simulink model "sim_tnse_2024_pos_ctrl"  (R2020a)
settings: Solver=ode4  StartTime=0.0  StopTime=30.0  FixedStep=0.01  RelTol=1e-3
values from neighbouring files (symbols this model uses):
  alfa_theta = 20    [init_tnse_2024_pos_ctrl.m]
  c1 = diag( [ 150.0, 120.0, 120.0 ] )    [init_tnse_2024_pos_ctrl.m]
  c1_diff_sigma_bar_v = diag([25; 30; 20])    [init_tnse_2024_pos_ctrl.m]
  c1v = diag([5.8; 6.5; 6.5])    [init_tnse_2024_pos_ctrl.m]
  c2 = diag( [ 80.0, 50.0, 50.0 ] )    [init_tnse_2024_pos_ctrl.m]
  c2_diff_sigma_bar_v = diag([50; 50; 10])    [init_tnse_2024_pos_ctrl.m]
  c2v = diag([5.8; 6.5; 6.5])    [init_tnse_2024_pos_ctrl.m]
  c3_diff_sigma_bar_v = diag([15; 15; 10])    [init_tnse_2024_pos_ctrl.m]
  c3v = diag([4.8; 6.4; 6.0])    [init_tnse_2024_pos_ctrl.m]
  dp_aa_t = 0.2 * ones(3, 5) + ( 1.0 - 0.2 ) * rand(3, 5)    [init_tnse_2024_pos_ctrl.m]
  dp_ff_t = [ 0.4 * ones(1, 5) + ( 1.0 - 0.4 ) * rand(1, 5);                      0.4 * ones(1, 5) + ( 1.0 - 0.4 ) * rand(1, 5);                      0.2 * ones(1, 5) + ( 0.6 - 0.2 ) * rand(1, 5) ]    [init_tnse_2024_pos_ctrl.m]
  dp_phi_t = ( - pi / 2 ) * ones(3, 5) + ( pi / 2 - ( - pi / 2 ) ) * rand(3, 5)    [init_tnse_2024_pos_ctrl.m]
  eps0 = [0.05; 0.01; 0.01]    [init_tnse_2024_pos_ctrl.m]
  etai_0 = zeros(3,5)    [init_tnse_2024_pos_ctrl.m]
  kai0 = [15; 10; 10]    [init_tnse_2024_pos_ctrl.m]
  kai_1_t = 0.02    [init_tnse_2024_pos_ctrl.m]
  kai_3_t = 0.1    [init_tnse_2024_pos_ctrl.m]
  ksii_0 = zeros(3,5)    [init_tnse_2024_pos_ctrl.m]
  lam0 = [15; 10; 10]    [init_tnse_2024_pos_ctrl.m]
  Lamd_diff_sigma_bar_v = 0.5    [init_tnse_2024_pos_ctrl.m]
  mass_i = zeros(1,NF)    [init_tnse_2024_pos_ctrl.m]
  Mii = diag([1;0;0;0;1])    [init_tnse_2024_pos_ctrl.m]
  pos0 = zeros(3, 1)    [init_tnse_2024_pos_ctrl.m]
  PZ0 = P0(3)    [init_tnse_2024_pos_ctrl.m]
  PZ1 = 10    [init_tnse_2024_pos_ctrl.m]
  Qci_init = repmat([1;0;0;0],1,NF)    [init_tnse_2024_pos_ctrl.m]
  R0 = 4    [init_tnse_2024_pos_ctrl.m]
  R1 = 8    [init_tnse_2024_pos_ctrl.m]
  Rx2 = 10    [init_tnse_2024_pos_ctrl.m]
  Ry2 = 6    [init_tnse_2024_pos_ctrl.m]
  Rz2 = 4    [init_tnse_2024_pos_ctrl.m]
  sat_sr_low = [-30, -30, -30]    [init_tnse_2024_pos_ctrl.m]
  sat_sr_up = [30, 30, 30]    [init_tnse_2024_pos_ctrl.m]
  T0 = 0    [init_tnse_2024_pos_ctrl.m]
  T1 = tseq1    (= 10)    [init_tnse_2024_pos_ctrl.m]
  T12 = tseq1 + tseq12    (= 20)    [init_tnse_2024_pos_ctrl.m]
  T2 = tseq1 + tseq12 + tseq2    (= 30)    [init_tnse_2024_pos_ctrl.m]
  theta0 = ( 2 / 5 ) * pi    (= 1.25663706144)    [init_tnse_2024_pos_ctrl.m]
  vel0 = zeros(3, 1)    [init_tnse_2024_pos_ctrl.m]
  Wij = [0,0,1,0,0;              0,0,1,1,0;              1,0,0,0,1;              0,1,1,0,0;              0,0,1,0,0]    [init_tnse_2024_pos_ctrl.m]
  X1 = 8    [init_tnse_2024_pos_ctrl.m]
  X2 = 2    [init_tnse_2024_pos_ctrl.m]
  X3 = 3    [init_tnse_2024_pos_ctrl.m]
  Y1 = 10    [init_tnse_2024_pos_ctrl.m]
  Y2 = 2    [init_tnse_2024_pos_ctrl.m]
  Y3 = 4    [init_tnse_2024_pos_ctrl.m]
  Z1 = 4    [init_tnse_2024_pos_ctrl.m]
  Z2 = -6    [init_tnse_2024_pos_ctrl.m]
  Z3 = 2    [init_tnse_2024_pos_ctrl.m]
  zeta_diff_sigma_bar_v = 0.08    [init_tnse_2024_pos_ctrl.m]
undefined symbols (not defined in the file or in its folder): cal_frac_squ, p_alfav1, p_alfav2, q_alfav1, q_alfav2
(part 1 of 4)
settings Model: Creator=zzy  LastModifiedBy=Hershey.A
settings DataIOCC: ReturnWorkspaceOutputs=off
settings DebuggingCC: ArithmeticOperatorsInVariantConditions=warning
settings SFSimCC: SimUseLocalCustomCode=off  CustomCodeUndefinedFunction=UseInterfaceOnly
settings RTWCC: RTWUseLocalCustomCode=off

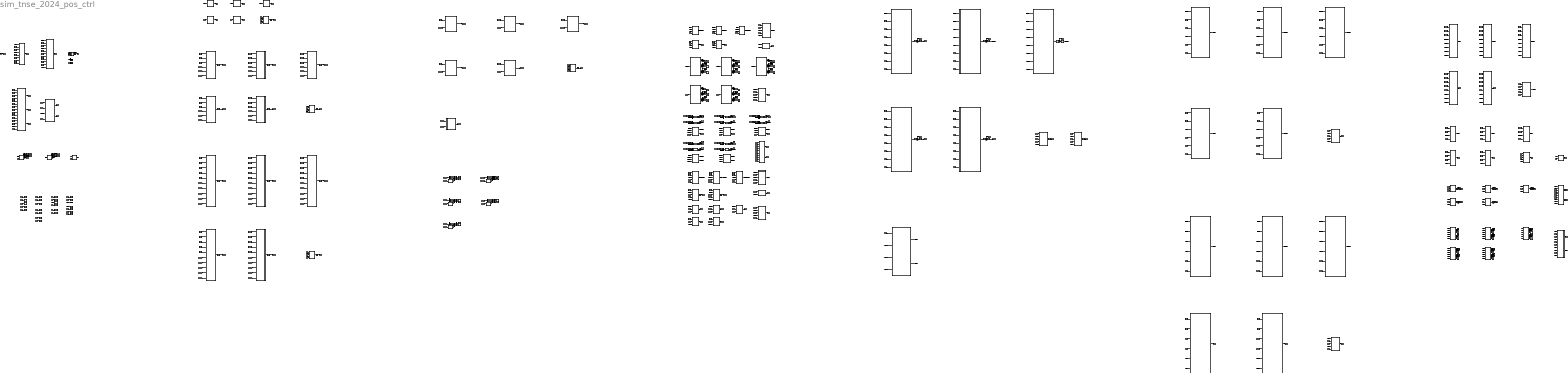
== system sim_tnse_2024_pos_ctrl ==
  Clock : Clock
  Constant{,3,6,9,14,17,22,27,32,37} (10 alike) : Constant  Value=eps0
  Constant{1,4,7,10,12,18,23,28,33,38,45,47,49,52,54,56,58,60..61,64,66,68,70,72,76} (25 alike) : Constant  Value=Wij
  Constant{100,102,107,112,117} (5 alike) : Constant  Value=p_alfav1
  Constant{101,103,108,113,118} (5 alike) : Constant  Value=alfa_theta
  Constant{97,104,109,114,119} (5 alike) : Constant  Value=q_alfav1
  Constant{98,105,110,115,120} (5 alike) : Constant  Value=p_alfav2
  Constant{99,106,111,116,121} (5 alike) : Constant  Value=q_alfav2
  Constant{2,5,8,11,13,19,24,29,34,39,46,48,50,53,55,57,59,62..63,65,67,69,71,73,77} (25 alike) : Constant  Value=Mii
  Constant{122,124,126,128,140} (5 alike) : Constant  Value=c1v
  Constant{123,125,127,139,141} (5 alike) : Constant  Value=c2v
  Constant{92..96,142..146} (10 alike) : Constant  Value=c3v
  Constant{88,147..148,152,157} (5 alike) : Constant  Value=sat_sr_low
  Constant{89,149,153,156,158} (5 alike) : Constant  Value=c2
  Constant{15,20,25,30,35} (5 alike) : Constant  Value=kai0
  Constant{86,90,150,154,159} (5 alike) : Constant  Value=c1
  Constant{87,91,151,155,160} (5 alike) : Constant  Value=sat_sr_up
  Constant{16,21,26,31,36,40..44} (10 alike) : Constant  Value=lam0
  Constant162 : Constant  Value=T1
  Constant163 : Constant  Value=R0
  Constant164 : Constant  Value=R1
  Constant165 : Constant  Value=T0
  Constant166 : Constant  Value=Rz2
  Constant167 : Constant  Value=Ry2
  Constant168 : Constant  Value=Rx2
  Constant169 : Constant  Value=X1
  Constant170 : Constant  Value=X2
  Constant171 : Constant  Value=Y1
  Constant172 : Constant  Value=Y2
  Constant173 : Constant  Value=T2
  Constant174 : Constant  Value=R0
  Constant175 : Constant  Value=R1
  Constant176 : Constant  Value=Rx2
  Constant177 : Constant  Value=Ry2
  Constant178 : Constant  Value=Rz2
  Constant179 : Constant  Value=T2
  Constant180 : Constant  Value=T1
  Constant181 : Constant  Value=PZ0
  Constant182 : Constant  Value=PZ1
  Constant191 : Constant  Value=mass_i
  Constant221 : Constant  Value=Z1
  Constant222 : Constant  Value=Z2
  Constant225 : Constant  Value=theta0
  Constant226 : Constant  Value=Z3
  Constant229 : Constant  Value=Y3
  Constant231 : Constant  Value=kai_1_t
  Constant234 : Constant  Value=X3
  Constant235 : Constant  Value=kai_3_t
  Constant238 : Constant  Value=T1
  Constant239 : Constant  Value=T12
  Constant{243,286,289,292,295} (5 alike) : Constant  Value=dp_phi_t
  Constant{244,287,290,293,296} (5 alike) : Constant  Value=dp_ff_t
  Constant{285,288,291,294,297} (5 alike) : Constant  Value=dp_aa_t
  Constant51 : Constant  Value=Qci_init
  Demux{1..10,12,22..33,38..45,94} (32 alike) : Demux  Outputs=3
  Display{6,12..25,35..59,64..68} (45 alike) : Display
  Interpreted MATLAB Function{20..29} (10 alike) : MATLABFcn  MATLABFcn=cal_frac_squ(u(1:3),u(4),u(5))
  Memory : Memory  InitialCondition=repmat(eye(3),1,1,5)
  Memory1 : Memory  InitialCondition=etai_0
  Memory2 : Memory  InitialCondition=ksii_0
  Memory{3,5..7} (4 alike) : Memory  InitialCondition=zeros(3,5)
  Memory4 : Memory  InitialCondition=zeros(1,5)
  Mux{1..12,133..135} (15 alike) : Mux  Inputs=2
  Mux{19..28} (10 alike) : Mux  Inputs=3
  Phi_sec_sigma_i agent 1 : MATLAB Function  TreatAsAtomicUnit=on
  Phi_sec_sigma_i agent 2 : MATLAB Function  TreatAsAtomicUnit=on
  Phi_sec_sigma_i agent 3 : MATLAB Function  TreatAsAtomicUnit=on
  Phi_sec_sigma_i agent 4 : MATLAB Function  TreatAsAtomicUnit=on
  Phi_sec_sigma_i agent 5 : MATLAB Function  TreatAsAtomicUnit=on
  Step : Step  Time=T1+0.01  SampleTime=0
  To Workspace : ToWorkspace  VariableName=sigmai  SampleTime=-1
  To Workspace1 : ToWorkspace  VariableName=dp_hat_vec  SampleTime=-1
  To Workspace10 : ToWorkspace  VariableName=eta_track_err_vec  SampleTime=-1
  To Workspace11 : ToWorkspace  VariableName=sigma_bar_v_hat_vec  SampleTime=-1
  To Workspace12 : ToWorkspace  VariableName=sigma_bar_v_vec  SampleTime=-1
  To Workspace13 : ToWorkspace  VariableName=sigma_bar_v_tilt_vec  SampleTime=-1
  To Workspace14 : ToWorkspace  VariableName=ui_vec  SampleTime=-1
  To Workspace15 : ToWorkspace  VariableName=rho_err  SampleTime=-1
  To Workspace16 : ToWorkspace  VariableName=psy  SampleTime=-1
  To Workspace17 : ToWorkspace  VariableName=rho_hat  SampleTime=-1
  To Workspace18 : ToWorkspace  VariableName=beta_hat  SampleTime=-1
  To Workspace19 : ToWorkspace  VariableName=sigma_v_vec  SampleTime=-1
  To Workspace2 : ToWorkspace  VariableName=dp_vec  SampleTime=-1
  To Workspace20 : ToWorkspace  VariableName=d_psy  SampleTime=-1
  To Workspace21 : ToWorkspace  VariableName=ri  SampleTime=-1
  To Workspace22 : ToWorkspace  VariableName=si  SampleTime=-1
  To Workspace23 : ToWorkspace  VariableName=delta_ksi_vec  SampleTime=-1
  To Workspace24 : ToWorkspace  VariableName=delta_eta_vec  SampleTime=-1
  To Workspace3 : ToWorkspace  VariableName=u0  SampleTime=-1
  To Workspace4 : ToWorkspace  VariableName=eta0  SampleTime=-1
  To Workspace5 : ToWorkspace  VariableName=ksi0  SampleTime=-1
  To Workspace6 : ToWorkspace  VariableName=dp_tilt_vec  SampleTime=-1
  To Workspace7 : ToWorkspace  VariableName=eta_i_vec  SampleTime=-1
  To Workspace8 : ToWorkspace  VariableName=ksi_i_vec  SampleTime=-1
  To Workspace9 : ToWorkspace  VariableName=ksi_track_err_vec  SampleTime=-1
  beta_hat Integrator {1..5} (5 alike) : Integrator
  cal Rci from ui : MATLAB Function  TreatAsAtomicUnit=on
  cal Rei : MATLAB Function  TreatAsAtomicUnit=on
  cal Ri : MATLAB Function  TreatAsAtomicUnit=on
  cal abs 21 : MATLAB Function  TreatAsAtomicUnit=on
  cal abs 22 : MATLAB Function  TreatAsAtomicUnit=on
  cal abs 23 : MATLAB Function  TreatAsAtomicUnit=on
  cal abs 24 : MATLAB Function  TreatAsAtomicUnit=on
  cal abs 25 : MATLAB Function  TreatAsAtomicUnit=on
  cal abs 26 : MATLAB Function  TreatAsAtomicUnit=on
  cal abs 27 : MATLAB Function  TreatAsAtomicUnit=on
  cal abs 28 : MATLAB Function  TreatAsAtomicUnit=on
  cal abs 29 : MATLAB Function  TreatAsAtomicUnit=on
  cal abs 30 : MATLAB Function  TreatAsAtomicUnit=on
  cal combine sigma_bar_v : MATLAB Function  TreatAsAtomicUnit=on
  cal combine sigma_bar_v_tilt : MATLAB Function  TreatAsAtomicUnit=on
  cal differentiator d_sigma_bar_v_hat agent 1 : Subsystem
  cal differentiator d_sigma_bar_v_hat agent 2 : Subsystem
  cal differentiator d_sigma_bar_v_hat agent 3 : Subsystem
  cal differentiator d_sigma_bar_v_hat agent 4 : Subsystem
  cal differentiator d_sigma_bar_v_hat agent 5 : Subsystem
  cal disturbance observation error dp_tilt : MATLAB Function  TreatAsAtomicUnit=on
  cal dp_hat agent 1 : MATLAB Function  TreatAsAtomicUnit=on
  cal dp_hat agent 2 : MATLAB Function  TreatAsAtomicUnit=on
  cal dp_hat agent 3 : MATLAB Function  TreatAsAtomicUnit=on
  cal dp_hat agent 4 : MATLAB Function  TreatAsAtomicUnit=on
  cal dp_hat agent 5 : MATLAB Function  TreatAsAtomicUnit=on
  cal eta_d_est ksi_d_est : MATLAB Function  TreatAsAtomicUnit=on
  cal rho_err_vec : MATLAB Function  TreatAsAtomicUnit=on
  cal ri agent 1 : MATLAB Function  TreatAsAtomicUnit=on
  cal ri agent 2 : MATLAB Function  TreatAsAtomicUnit=on
  cal ri agent 3 : MATLAB Function  TreatAsAtomicUnit=on
  cal ri agent 4 : MATLAB Function  TreatAsAtomicUnit=on
  cal ri agent 5 : MATLAB Function  TreatAsAtomicUnit=on
  cal si agent 1 : MATLAB Function  TreatAsAtomicUnit=on
  cal si agent 2 : MATLAB Function  TreatAsAtomicUnit=on
  cal si agent 3 : MATLAB Function  TreatAsAtomicUnit=on
  cal si agent 4 : MATLAB Function  TreatAsAtomicUnit=on
  cal si agent 5 : MATLAB Function  TreatAsAtomicUnit=on
  cal sigma_bar_v_hat agent 1 : MATLAB Function  TreatAsAtomicUnit=on
  cal sigma_bar_v_hat agent 2 : MATLAB Function  TreatAsAtomicUnit=on
  cal sigma_bar_v_hat agent 3 : MATLAB Function  TreatAsAtomicUnit=on
  cal sigma_bar_v_hat agent 4 : MATLAB Function  TreatAsAtomicUnit=on
  cal sigma_bar_v_hat agent 5 : MATLAB Function  TreatAsAtomicUnit=on
  cal theta_sigma_bar_v_tilt agent 1 : MATLAB Function  TreatAsAtomicUnit=on
  cal theta_sigma_bar_v_tilt agent 2 : MATLAB Function  TreatAsAtomicUnit=on
  cal theta_sigma_bar_v_tilt agent 3 : MATLAB Function  TreatAsAtomicUnit=on
  cal theta_sigma_bar_v_tilt agent 4 : MATLAB Function  TreatAsAtomicUnit=on
  cal theta_sigma_bar_v_tilt agent 5 : MATLAB Function  TreatAsAtomicUnit=on
  cal ui agent 1 : MATLAB Function  TreatAsAtomicUnit=on
  cal ui agent 2 : MATLAB Function  TreatAsAtomicUnit=on
  cal ui agent 3 : MATLAB Function  TreatAsAtomicUnit=on
  cal ui agent 4 : MATLAB Function  TreatAsAtomicUnit=on
  cal ui agent 5 : MATLAB Function  TreatAsAtomicUnit=on
  cal virtual control sigma_v agent 1 : MATLAB Function  TreatAsAtomicUnit=on
  cal virtual control sigma_v agent 2 : MATLAB Function  TreatAsAtomicUnit=on
  cal virtual control sigma_v agent 3 : MATLAB Function  TreatAsAtomicUnit=on
  cal virtual control sigma_v agent 4 : MATLAB Function  TreatAsAtomicUnit=on
  cal virtual control sigma_v agent 5 : MATLAB Function  TreatAsAtomicUnit=on
  choose ksi_est_err 21 : MATLAB Function  TreatAsAtomicUnit=on
  choose ksi_est_err 22 : MATLAB Function  TreatAsAtomicUnit=on
  choose ksi_est_err 23 : MATLAB Function  TreatAsAtomicUnit=on
  choose ksi_est_err 24 : MATLAB Function  TreatAsAtomicUnit=on
  choose ksi_est_err 25 : MATLAB Function  TreatAsAtomicUnit=on
  choose ksi_est_err 26 : MATLAB Function  TreatAsAtomicUnit=on
  choose ksi_est_err 27 : MATLAB Function  TreatAsAtomicUnit=on
  choose ksi_est_err 28 : MATLAB Function  TreatAsAtomicUnit=on
  choose ksi_est_err 29 : MATLAB Function  TreatAsAtomicUnit=on
  choose ksi_est_err 30 : MATLAB Function  TreatAsAtomicUnit=on
  choose rho_hat agent 1 : MATLAB Function  TreatAsAtomicUnit=on
  choose rho_hat agent 2 : MATLAB Function  TreatAsAtomicUnit=on
  choose rho_hat agent 3 : MATLAB Function  TreatAsAtomicUnit=on
  choose rho_hat agent 4 : MATLAB Function  TreatAsAtomicUnit=on
  choose rho_hat agent 5 : MATLAB Function  TreatAsAtomicUnit=on
  combine Phi_sec_sigma_i : MATLAB Function  TreatAsAtomicUnit=on
  combine betai : MATLAB Function  TreatAsAtomicUnit=on
  combine betai1 : MATLAB Function  TreatAsAtomicUnit=on
  combine d_psy : MATLAB Function  TreatAsAtomicUnit=on
  combine d_sigma_bar_v_est : MATLAB Function  TreatAsAtomicUnit=on
  combine dp_hat : MATLAB Function  TreatAsAtomicUnit=on
  combine follower eta ksi : MATLAB Function  TreatAsAtomicUnit=on
  combine formation control input : MATLAB Function  TreatAsAtomicUnit=on
  combine psy : MATLAB Function  TreatAsAtomicUnit=on
  combine rho_hat : MATLAB Function  TreatAsAtomicUnit=on
  combine ri : MATLAB Function  TreatAsAtomicUnit=on
  combine si : MATLAB Function  TreatAsAtomicUnit=on
  combine sigma_bar_v_hat : MATLAB Function  TreatAsAtomicUnit=on
  combine sigma_v : MATLAB Function  TreatAsAtomicUnit=on
  combine theta_sigma_bar_v_tilt : MATLAB Function  TreatAsAtomicUnit=on
  combine translational disturbance : MATLAB Function  TreatAsAtomicUnit=on
  combine ui : MATLAB Function  TreatAsAtomicUnit=on
  d2_sigma_bar_v_est_{1..5} (5 alike) : Scope  NumInputPorts=3
  d_psy Integrator {1..5} (5 alike) : Integrator  InitialCondition=zeros(3,1)
  d_sigma_bar_v_est_{1..5} (5 alike) : Scope  NumInputPorts=3
  depart Rc1 : MATLAB Function  TreatAsAtomicUnit=on
  depart Rc2 : MATLAB Function  TreatAsAtomicUnit=on
  depart Rc3 : MATLAB Function  TreatAsAtomicUnit=on
  depart Rc4 : MATLAB Function  TreatAsAtomicUnit=on
  depart Rc5 : MATLAB Function  TreatAsAtomicUnit=on
  depart Re1 : MATLAB Function  TreatAsAtomicUnit=on
  depart Re2 : MATLAB Function  TreatAsAtomicUnit=on
  depart Re3 : MATLAB Function  TreatAsAtomicUnit=on
  depart Re4 : MATLAB Function  TreatAsAtomicUnit=on
  depart Re5 : MATLAB Function  TreatAsAtomicUnit=on
  desire formation position and velocity : MATLAB Function  TreatAsAtomicUnit=on
  eta_0 : Scope  NumInputPorts=3
  eta_track_err_{1..5} (5 alike) : Scope  NumInputPorts=3
  follower etai Integrator agent 1 : Integrator  InitialCondition=etai_0(:,1)
  follower etai Integrator agent 2 : Integrator  InitialCondition=etai_0(:,2)
  follower etai Integrator agent 3 : Integrator  InitialCondition=etai_0(:,3)
  follower etai Integrator agent 4 : Integrator  InitialCondition=etai_0(:,4)
  follower etai Integrator agent 5 : Integrator  InitialCondition=etai_0(:,5)
  follower ksii Integrator agent 1 : Integrator  InitialCondition=ksii_0(:,1)
  follower ksii Integrator agent 2 : Integrator  InitialCondition=ksii_0(:,2)
  follower ksii Integrator agent 3 : Integrator  InitialCondition=ksii_0(:,3)
  follower ksii Integrator agent 4 : Integrator  InitialCondition=ksii_0(:,4)
  follower ksii Integrator agent 5 : Integrator  InitialCondition=ksii_0(:,5)
  follower tracking error agent 1 : MATLAB Function  TreatAsAtomicUnit=on
  follower tracking error agent 2 : MATLAB Function  TreatAsAtomicUnit=on
  follower tracking error agent 3 : MATLAB Function  TreatAsAtomicUnit=on
  follower tracking error agent 4 : MATLAB Function  TreatAsAtomicUnit=on
  follower tracking error agent 5 : MATLAB Function  TreatAsAtomicUnit=on
  generate translational disturbance agent 1 : MATLAB Function  TreatAsAtomicUnit=on
  generate translational disturbance agent 2 : MATLAB Function  TreatAsAtomicUnit=on
  generate translational disturbance agent 3 : MATLAB Function  TreatAsAtomicUnit=on
  generate translational disturbance agent 4 : MATLAB Function  TreatAsAtomicUnit=on
  generate translational disturbance agent 5 : MATLAB Function  TreatAsAtomicUnit=on
  ksi_0 : Scope  NumInputPorts=3
  ksi_track_err_{1..5} (5 alike) : Scope  NumInputPorts=3
  leader control input : MATLAB Function  TreatAsAtomicUnit=on
  leader eta0 Integrator : Integrator  ExternalReset=rising  InitialConditionSource=external  InitialCondition=vel0
  leader ksi0 Integrator : Integrator  InitialCondition=pos0
  process velocity : MATLAB Function  TreatAsAtomicUnit=on
  psy Integrator {1..5} (5 alike) : Integrator  InitialCondition=zeros(3,1)
  rho_hat agent 1 : MATLAB Function  TreatAsAtomicUnit=on
  rho_hat agent 2 : MATLAB Function  TreatAsAtomicUnit=on
  rho_hat agent 3 : MATLAB Function  TreatAsAtomicUnit=on
  rho_hat agent 4 : MATLAB Function  TreatAsAtomicUnit=on
  rho_hat agent 5 : MATLAB Function  TreatAsAtomicUnit=on
  set desire formation configuration : MATLAB Function  TreatAsAtomicUnit=on
  sigma_bar_v_hat Integrator {1..5} (5 alike) : Integrator  InitialCondition=zeros(3,1)
  sigma_v Integrator {1..5} (5 alike) : Integrator  InitialCondition=zeros(3,1)
  sigmai Integrator {1..5} (5 alike) : Integrator  InitialCondition=zeros(3,1)
  trans to column20 : MATLAB Function  TreatAsAtomicUnit=on
  trans to column21 : MATLAB Function  TreatAsAtomicUnit=on
  trans to column22 : MATLAB Function  TreatAsAtomicUnit=on
  trans to column23 : MATLAB Function  TreatAsAtomicUnit=on
  trans to column24 : MATLAB Function  TreatAsAtomicUnit=on
  trans to column25 : MATLAB Function  TreatAsAtomicUnit=on
  trans to column26 : MATLAB Function  TreatAsAtomicUnit=on
  trans to column27 : MATLAB Function  TreatAsAtomicUnit=on
  trans to column28 : MATLAB Function  TreatAsAtomicUnit=on
  trans to column29 : MATLAB Function  TreatAsAtomicUnit=on
  u0 vs rho_hat agent {1..5} (5 alike) : Scope  NumInputPorts=3
  uav translational dynamics agent 1 : MATLAB Function  TreatAsAtomicUnit=on
  uav translational dynamics agent 2 : MATLAB Function  TreatAsAtomicUnit=on
  uav translational dynamics agent 3 : MATLAB Function  TreatAsAtomicUnit=on
  uav translational dynamics agent 4 : MATLAB Function  TreatAsAtomicUnit=on
  uav translational dynamics agent 5 : MATLAB Function  TreatAsAtomicUnit=on
  update betai agent 1 : MATLAB Function  TreatAsAtomicUnit=on
  update betai agent 2 : MATLAB Function  TreatAsAtomicUnit=on
  update betai agent 3 : MATLAB Function  TreatAsAtomicUnit=on
  update betai agent 4 : MATLAB Function  TreatAsAtomicUnit=on
  update betai agent 5 : MATLAB Function  TreatAsAtomicUnit=on
  update dpsy psy agent 1 : MATLAB Function  TreatAsAtomicUnit=on
  update dpsy psy agent 2 : MATLAB Function  TreatAsAtomicUnit=on
  update dpsy psy agent 3 : MATLAB Function  TreatAsAtomicUnit=on
  update dpsy psy agent 4 : MATLAB Function  TreatAsAtomicUnit=on
  update dpsy psy agent 5 : MATLAB Function  TreatAsAtomicUnit=on
  update sigmai agent 1 : MATLAB Function  TreatAsAtomicUnit=on
  update sigmai agent 2 : MATLAB Function  TreatAsAtomicUnit=on
  update sigmai agent 3 : MATLAB Function  TreatAsAtomicUnit=on
  update sigmai agent 4 : MATLAB Function  TreatAsAtomicUnit=on
  update sigmai agent 5 : MATLAB Function  TreatAsAtomicUnit=on
  wires:
  follower etai Integrator agent 1/1 -> [eta_1], follower ksii Integrator agent 1/1
  follower etai Integrator agent 2/1 -> [eta_2], follower ksii Integrator agent 2/1
  follower etai Integrator agent 3/1 -> [eta_3], follower ksii Integrator agent 3/1
  follower etai Integrator agent 4/1 -> [eta_4], follower ksii Integrator agent 4/1
  follower etai Integrator agent 5/1 -> [eta_5], follower ksii Integrator agent 5/1
  follower ksii Integrator agent 1/1 -> [ksi_1]
  follower ksii Integrator agent 2/1 -> [ksi_2]
  follower ksii Integrator agent 3/1 -> [ksi_3]
  follower ksii Integrator agent 4/1 -> [ksi_4]
  follower ksii Integrator agent 5/1 -> [ksi_5]
  [eta_1] -> combine formation control input/1(eta_1)
  [eta_2] -> combine formation control input/2(eta_2)
  [eta_3] -> combine formation control input/3(eta_3)
  [eta_4] -> combine formation control input/4(eta_4)
  [eta_5] -> combine formation control input/5(eta_5)
  [ksi_1] -> combine formation control input/6(ksi_1)
  [ksi_2] -> combine formation control input/7(ksi_2)
  [ksi_3] -> combine formation control input/8(ksi_3)
  [ksi_4] -> combine formation control input/9(ksi_4)
  [ksi_5] -> combine formation control input/10(ksi_5)
  [ksi_i_vec] -> follower tracking error agent 1/3(ksi_i_vec)
  [eta_i_vec] -> follower tracking error agent 1/4(eta_i_vec)
  [ksi0] -> follower tracking error agent 1/5(ksi0)
  [eta0] -> follower tracking error agent 1/6(eta0)
  follower tracking error agent 1/2(eta_track_err_1) -> Display13/1, Demux24/1, [eta_track_err_1]
  follower tracking error agent 1/1(ksi_track_err_1) -> Display12/1, Demux23/1, [ksi_track_err_1]
  [eta0] -> follower tracking error agent 2/6(eta0)
  [ksi0] -> follower tracking error agent 2/5(ksi0)
  [eta_i_vec] -> follower tracking error agent 2/4(eta_i_vec)
  follower tracking error agent 2/2(eta_track_err_2) -> Display15/1, Demux26/1, [eta_track_err_2]
  [ksi_i_vec] -> follower tracking error agent 2/3(ksi_i_vec)
  follower tracking error agent 2/1(ksi_track_err_2) -> Display14/1, Demux25/1, [ksi_track_err_2]
  follower tracking error agent 3/2(eta_track_err_3) -> Display17/1, Demux28/1, [eta_track_err_3]
  follower tracking error agent 3/1(ksi_track_err_3) -> Display16/1, Demux27/1, [ksi_track_err_3]
  [eta0] -> follower tracking error agent 3/6(eta0)
  [eta_i_vec] -> follower tracking error agent 3/4(eta_i_vec)
  [ksi_i_vec] -> follower tracking error agent 3/3(ksi_i_vec)
  [ksi0] -> follower tracking error agent 3/5(ksi0)
  [ksi_i_vec] -> follower tracking error agent 4/3(ksi_i_vec)
  [ksi0] -> follower tracking error agent 4/5(ksi0)
  [eta_i_vec] -> follower tracking error agent 4/4(eta_i_vec)
  [eta0] -> follower tracking error agent 4/6(eta0)
  follower tracking error agent 4/2(eta_track_err_4) -> Display19/1, Demux30/1, [eta_track_err_4]
  follower tracking error agent 4/1(ksi_track_err_4) -> Display18/1, Demux29/1, [ksi_track_err_4]
  follower tracking error agent 5/1(ksi_track_err_5) -> Display20/1, Demux31/1, [ksi_track_err_5]
  [ksi_i_vec] -> follower tracking error agent 5/3(ksi_i_vec)
  [eta0] -> follower tracking error agent 5/6(eta0)
  [ksi0] -> follower tracking error agent 5/5(ksi0)
  [eta_i_vec] -> follower tracking error agent 5/4(eta_i_vec)
  follower tracking error agent 5/2(eta_track_err_5) -> Display21/1, Demux32/1, [eta_track_err_5]
  [ksi_track_err_1] -> combine follower eta ksi/1(ksi_track_err_1)
  [ksi_track_err_2] -> combine follower eta ksi/2(ksi_track_err_2)
  [ksi_track_err_3] -> combine follower eta ksi/3(ksi_track_err_3)
  [ksi_track_err_4] -> combine follower eta ksi/4(ksi_track_err_4)
  [ksi_track_err_5] -> combine follower eta ksi/5(ksi_track_err_5)
  [eta_track_err_1] -> combine follower eta ksi/6(eta_track_err_1)
  [eta_track_err_2] -> combine follower eta ksi/7(eta_track_err_2)
  [eta_track_err_3] -> combine follower eta ksi/8(eta_track_err_3)
  [eta_track_err_4] -> combine follower eta ksi/9(eta_track_err_4)
  [eta_track_err_5] -> combine follower eta ksi/10(eta_track_err_5)
  combine follower eta ksi/1(ksi_track_err_vec) -> [ksi_track_err_vec]
  combine follower eta ksi/2(eta_track_err_vec) -> [eta_track_err_vec]
  Demux23/2 -> ksi_track_err_1/2
  Demux23/1 -> ksi_track_err_1/1
  Demux23/3 -> ksi_track_err_1/3
  Demux24/2 -> eta_track_err_1/2
  Demux24/1 -> eta_track_err_1/1
  Demux24/3 -> eta_track_err_1/3
  Demux25/2 -> ksi_track_err_2/2
  Demux25/1 -> ksi_track_err_2/1
  Demux25/3 -> ksi_track_err_2/3
  Demux26/1 -> eta_track_err_2/1
  Demux26/3 -> eta_track_err_2/3
  Demux26/2 -> eta_track_err_2/2
  Demux27/1 -> ksi_track_err_3/1
  Demux27/3 -> ksi_track_err_3/3
  Demux27/2 -> ksi_track_err_3/2
  Demux28/3 -> eta_track_err_3/3
  Demux28/2 -> eta_track_err_3/2
  Demux28/1 -> eta_track_err_3/1
  Demux29/3 -> ksi_track_err_4/3
  Demux29/2 -> ksi_track_err_4/2
  Demux29/1 -> ksi_track_err_4/1
  Demux30/3 -> eta_track_err_4/3
  Demux30/2 -> eta_track_err_4/2
  Demux30/1 -> eta_track_err_4/1
  Demux31/3 -> ksi_track_err_5/3
  Demux31/2 -> ksi_track_err_5/2
  Demux31/1 -> ksi_track_err_5/1
  Demux32/3 -> eta_track_err_5/3
  Demux32/2 -> eta_track_err_5/2
  Demux32/1 -> eta_track_err_5/1
  combine formation control input/1(eta_i_vec) -> Memory1/1
  Memory1/1 -> [eta_i_vec]
  combine formation control input/2(ksi_i_vec) -> Memory2/1
  Memory2/1 -> [ksi_i_vec]
  [ui] -> uav translational dynamics agent 1/2(ui_vec)
  [Ri] -> uav translational dynamics agent 1/1(Ri)
  uav translational dynamics agent 1/1(dvi) -> follower etai Integrator agent 1/1
  uav translational dynamics agent 2/1(dvi) -> follower etai Integrator agent 2/1
  [ui] -> uav translational dynamics agent 2/2(ui_vec)
  [Ri] -> uav translational dynamics agent 2/1(Ri)
  [ui] -> uav translational dynamics agent 3/2(ui_vec)
  [Ri] -> uav translational dynamics agent 3/1(Ri)
  uav translational dynamics agent 3/1(dvi) -> follower etai Integrator agent 3/1
  [ui] -> uav translational dynamics agent 4/2(ui_vec)
  [Ri] -> uav translational dynamics agent 4/1(Ri)
  uav translational dynamics agent 4/1(dvi) -> follower etai Integrator agent 4/1
  [ui] -> uav translational dynamics agent 5/2(ui_vec)
  [Ri] -> uav translational dynamics agent 5/1(Ri)
  uav translational dynamics agent 5/1(dvi) -> follower etai Integrator agent 5/1
  [ui] -> cal Rci from ui/2(ui_vec)
  Constant191/1 -> cal Rci from ui/1(mi_vec)
  cal Rei/1(Rei) -> depart Re5/1(x), depart Re4/1(x), depart Re3/1(x), depart Re2/1(x), depart Re1/1(x), [Rei]
  depart Re2/1(y) -> Display65/1
  depart Re3/1(y) -> Display66/1
  depart Re1/1(y) -> Display64/1
  depart Re4/1(y) -> Display67/1
  Constant51/1 -> cal Rei/1(Qei)
  depart Re5/1(y) -> Display68/1
  [Rei] -> cal Ri/1(Rei)
  [Rci] -> cal Ri/2(Rci)
  cal Ri/1(Ri) -> [Ri]
  depart Rc5/1(y) -> Display25/1
  depart Rc2/1(y) -> Display22/1
  depart Rc3/1(y) -> Display23/1
  depart Rc4/1(y) -> Display24/1
  depart Rc1/1(y) -> Display6/1
  cal Rci from ui/1(Rci) -> [Rci], depart Rc5/1(x), depart Rc4/1(x), depart Rc3/1(x), depart Rc2/1(x), depart Rc1/1(x)
  [dp_vec] -> uav translational dynamics agent 1/3(dpi_vec)
  [dp_vec] -> uav translational dynamics agent 2/3(dpi_vec)
  [dp_vec] -> uav translational dynamics agent 3/3(dpi_vec)
  [dp_vec] -> uav translational dynamics agent 4/3(dpi_vec)
  [dp_vec] -> uav translational dynamics agent 5/3(dpi_vec)
  [Ri] -> cal virtual control sigma_v agent 1/2(Ri)
  [ui] -> cal virtual control sigma_v agent 1/3(ui_vec)
  Constant92/1 -> cal virtual control sigma_v agent 1/1(c3v)
  [sigma_bar_v_vec] -> cal virtual control sigma_v agent 1/4(sigma_bar_v_vec)
  cal virtual control sigma_v agent 1/1(d_sigma_v_1) -> sigma_v Integrator 1/1
  sigma_v Integrator 1/1 -> [sigma_v_1]
  [sigma_bar_v_vec] -> cal virtual control sigma_v agent 2/4(sigma_bar_v_vec)
  sigma_v Integrator 2/1 -> [sigma_v_2]
  Constant93/1 -> cal virtual control sigma_v agent 2/1(c3v)
  [Ri] -> cal virtual control sigma_v agent 2/2(Ri)
  cal virtual control sigma_v agent 2/1(d_sigma_v_2) -> sigma_v Integrator 2/1
  [ui] -> cal virtual control sigma_v agent 2/3(ui_vec)
  Constant94/1 -> cal virtual control sigma_v agent 3/1(c3v)
  cal virtual control sigma_v agent 3/1(d_sigma_v_3) -> sigma_v Integrator 3/1
  [ui] -> cal virtual control sigma_v agent 3/3(ui_vec)
  [Ri] -> cal virtual control sigma_v agent 3/2(Ri)
  [sigma_bar_v_vec] -> cal virtual control sigma_v agent 3/4(sigma_bar_v_vec)
  sigma_v Integrator 3/1 -> [sigma_v_3]
  sigma_v Integrator 4/1 -> [sigma_v_4]
  [Ri] -> cal virtual control sigma_v agent 4/2(Ri)
  [sigma_bar_v_vec] -> cal virtual control sigma_v agent 4/4(sigma_bar_v_vec)
  [ui] -> cal virtual control sigma_v agent 4/3(ui_vec)
  cal virtual control sigma_v agent 4/1(d_sigma_v_4) -> sigma_v Integrator 4/1
  Constant95/1 -> cal virtual control sigma_v agent 4/1(c3v)
  Constant96/1 -> cal virtual control sigma_v agent 5/1(c3v)
  [sigma_bar_v_vec] -> cal virtual control sigma_v agent 5/4(sigma_bar_v_vec)
  [Ri] -> cal virtual control sigma_v agent 5/2(Ri)
  [ui] -> cal virtual control sigma_v agent 5/3(ui_vec)
  sigma_v Integrator 5/1 -> [sigma_v_5]
  cal virtual control sigma_v agent 5/1(d_sigma_v_5) -> sigma_v Integrator 5/1
  combine sigma_v/1(sigma_v_vec) -> [sigma_v_vec]
  [sigma_v_4] -> combine sigma_v/4(sigma_v_4)
  [sigma_v_3] -> combine sigma_v/3(sigma_v_3)
  [sigma_v_1] -> combine sigma_v/1(sigma_v_1)
  [sigma_v_5] -> combine sigma_v/5(sigma_v_5)
  [sigma_v_2] -> combine sigma_v/2(sigma_v_2)
  [eta_i_vec] -> cal combine sigma_bar_v/1(eta_i_vec)
  [sigma_v_vec] -> cal combine sigma_bar_v/2(sigma_v_vec)
  cal combine sigma_bar_v/1(sigma_bar_v_vec) -> [sigma_bar_v_vec]
  Demux12/3 -> d2_sigma_bar_v_est_1/3
  Demux12/2 -> d2_sigma_bar_v_est_1/2
  Demux8/3 -> d_sigma_bar_v_est_1/3
  Demux12/1 -> d2_sigma_bar_v_est_1/1
  Demux8/1 -> d_sigma_bar_v_est_1/1
  Demux8/2 -> d_sigma_bar_v_est_1/2
  cal differentiator d_sigma_bar_v_hat agent 1/1(Out1) -> Display35/1, [sigma_bar_v_est_1]
  cal differentiator d_sigma_bar_v_hat agent 1/2(Out2) -> Demux8/1, [d_sigma_bar_v_est_1], Display36/1
  cal differentiator d_sigma_bar_v_hat agent 1/3(Out3) -> Demux12/1, [d2_sigma_bar_v_est_1], Display37/1
  [sigma_bar_v_vec] -> cal differentiator d_sigma_bar_v_hat agent 1/1(x)
  cal differentiator d_sigma_bar_v_hat agent 2/1(Out1) -> Display38/1, [sigma_bar_v_est_2]
  [sigma_bar_v_vec] -> cal differentiator d_sigma_bar_v_hat agent 2/1(x)
  cal differentiator d_sigma_bar_v_hat agent 2/2(Out2) -> Demux3/1, [d_sigma_bar_v_est_2], Display39/1
  cal differentiator d_sigma_bar_v_hat agent 2/3(Out3) -> Demux2/1, [d2_sigma_bar_v_est_2], Display40/1
  Demux2/2 -> d2_sigma_bar_v_est_2/2
  Demux2/3 -> d2_sigma_bar_v_est_2/3
  Demux3/2 -> d_sigma_bar_v_est_2/2
  Demux2/1 -> d2_sigma_bar_v_est_2/1
  Demux3/1 -> d_sigma_bar_v_est_2/1
  Demux3/3 -> d_sigma_bar_v_est_2/3
  Demux5/1 -> d_sigma_bar_v_est_3/1
  Demux5/3 -> d_sigma_bar_v_est_3/3
  Demux4/2 -> d2_sigma_bar_v_est_3/2
  Demux4/3 -> d2_sigma_bar_v_est_3/3
  Demux5/2 -> d_sigma_bar_v_est_3/2
  Demux4/1 -> d2_sigma_bar_v_est_3/1
  cal differentiator d_sigma_bar_v_hat agent 3/3(Out3) -> Demux4/1, [d2_sigma_bar_v_est_3], Display43/1
  cal differentiator d_sigma_bar_v_hat agent 3/2(Out2) -> Demux5/1, [d_sigma_bar_v_est_3], Display42/1
  cal differentiator d_sigma_bar_v_hat agent 3/1(Out1) -> Display41/1, [sigma_bar_v_est_3]
  [sigma_bar_v_vec] -> cal differentiator d_sigma_bar_v_hat agent 3/1(x)
  cal differentiator d_sigma_bar_v_hat agent 4/3(Out3) -> Demux6/1, [d2_sigma_bar_v_est_4], Display46/1
  Demux6/1 -> d2_sigma_bar_v_est_4/1
  Demux6/3 -> d2_sigma_bar_v_est_4/3
  Demux7/2 -> d_sigma_bar_v_est_4/2
  Demux6/2 -> d2_sigma_bar_v_est_4/2
  Demux7/3 -> d_sigma_bar_v_est_4/3
  Demux7/1 -> d_sigma_bar_v_est_4/1
  cal differentiator d_sigma_bar_v_hat agent 4/1(Out1) -> Display44/1, [sigma_bar_v_est_4]
  cal differentiator d_sigma_bar_v_hat agent 4/2(Out2) -> Demux7/1, [d_sigma_bar_v_est_4], Display45/1
  [sigma_bar_v_vec] -> cal differentiator d_sigma_bar_v_hat agent 4/1(x)
  cal differentiator d_sigma_bar_v_hat agent 5/1(Out1) -> Display47/1, [sigma_bar_v_est_5]
  cal differentiator d_sigma_bar_v_hat agent 5/2(Out2) -> Demux10/1, [d_sigma_bar_v_est_5], Display48/1
  [sigma_bar_v_vec] -> cal differentiator d_sigma_bar_v_hat agent 5/1(x)
  Demux10/3 -> d_sigma_bar_v_est_5/3
  Demux9/2 -> d2_sigma_bar_v_est_5/2
  Demux10/2 -> d_sigma_bar_v_est_5/2
  Demux9/1 -> d2_sigma_bar_v_est_5/1
  cal differentiator d_sigma_bar_v_hat agent 5/3(Out3) -> Demux9/1, [d2_sigma_bar_v_est_5], Display49/1
  Demux10/1 -> d_sigma_bar_v_est_5/1
  Demux9/3 -> d2_sigma_bar_v_est_5/3
  [d_sigma_bar_v_est_5] -> combine d_sigma_bar_v_est/5(d_sigma_bar_v_est_5)
  [d_sigma_bar_v_est_2] -> combine d_sigma_bar_v_est/2(d_sigma_bar_v_est_2)
  [d_sigma_bar_v_est_1] -> combine d_sigma_bar_v_est/1(d_sigma_bar_v_est_1)
  [d_sigma_bar_v_est_4] -> combine d_sigma_bar_v_est/4(d_sigma_bar_v_est_4)
  [d_sigma_bar_v_est_3] -> combine d_sigma_bar_v_est/3(d_sigma_bar_v_est_3)
  combine d_sigma_bar_v_est/1(d_sigma_bar_v_vec) -> [d_sigma_bar_v_vec]
  trans to column21/1(y) -> [sigma_bar_v_tilt_squ_1_1], Display51/1
  Constant100/1 -> Mux20/2
  Constant97/1 -> Mux20/3
  Interpreted MATLAB Function21/1 -> trans to column21/1(x)
  [sigma_bar_v_tilt_vec] -> choose ksi_est_err 21/1(x)
  choose ksi_est_err 21/1(y) -> cal abs 21/1(x)
  Constant98/1 -> Mux19/2
  cal abs 22/1(y) -> Mux19/1
  choose ksi_est_err 22/1(y) -> cal abs 22/1(x)
  Interpreted MATLAB Function20/1 -> trans to column20/1(x)
  cal abs 21/1(y) -> Mux20/1
  Mux19/1 -> Interpreted MATLAB Function20/1
  trans to column20/1(y) -> [sigma_bar_v_tilt_squ_2_1], Display50/1
  Constant99/1 -> Mux19/3
  Mux20/1 -> Interpreted MATLAB Function21/1
  [sigma_bar_v_tilt_vec] -> choose ksi_est_err 22/1(x)
  cal theta_sigma_bar_v_tilt agent 1/1(theta_sigma_bar_v_tilt_1_1) -> [theta_sigma_bar_v_tilt_1_1]
  [sigma_bar_v_tilt_squ_1_1] -> cal theta_sigma_bar_v_tilt agent 1/2(sigma_bar_v_tilt_squ_1_1)
  cal theta_sigma_bar_v_tilt agent 1/2(theta_sigma_bar_v_tilt_2_1) -> [theta_sigma_bar_v_tilt_2_1]
  [sigma_bar_v_tilt_vec] -> cal theta_sigma_bar_v_tilt agent 1/4(sigma_bar_v_tilt_vec)
  [sigma_bar_v_tilt_squ_2_1] -> cal theta_sigma_bar_v_tilt agent 1/3(sigma_bar_v_tilt_squ_2_1)
  Constant101/1 -> cal theta_sigma_bar_v_tilt agent 1/1(alfa_theta)
  Constant103/1 -> cal theta_sigma_bar_v_tilt agent 2/1(alfa_theta)
  [sigma_bar_v_tilt_vec] -> cal theta_sigma_bar_v_tilt agent 2/4(sigma_bar_v_tilt_vec)
  [sigma_bar_v_tilt_squ_1_2] -> cal theta_sigma_bar_v_tilt agent 2/2(sigma_bar_v_tilt_squ_1_2)
  trans to column23/1(y) -> [sigma_bar_v_tilt_squ_1_2], Display53/1
  Interpreted MATLAB Function23/1 -> trans to column23/1(x)
  Mux22/1 -> Interpreted MATLAB Function23/1
  Constant106/1 -> Mux21/3
  cal theta_sigma_bar_v_tilt agent 2/1(theta_sigma_bar_v_tilt_1_2) -> [theta_sigma_bar_v_tilt_1_2]
  Constant102/1 -> Mux22/2
  trans to column22/1(y) -> [sigma_bar_v_tilt_squ_2_2], Display52/1
  Interpreted MATLAB Function22/1 -> trans to column22/1(x)
  cal abs 23/1(y) -> Mux22/1
  Constant104/1 -> Mux22/3
  Mux21/1 -> Interpreted MATLAB Function22/1
  choose ksi_est_err 24/1(y) -> cal abs 24/1(x)
  cal abs 24/1(y) -> Mux21/1
  choose ksi_est_err 23/1(y) -> cal abs 23/1(x)
  [sigma_bar_v_tilt_vec] -> choose ksi_est_err 24/1(x)
  [sigma_bar_v_tilt_squ_2_2] -> cal theta_sigma_bar_v_tilt agent 2/3(sigma_bar_v_tilt_squ_2_2)
  Constant105/1 -> Mux21/2
  [sigma_bar_v_tilt_vec] -> choose ksi_est_err 23/1(x)
  cal theta_sigma_bar_v_tilt agent 2/2(theta_sigma_bar_v_tilt_2_2) -> [theta_sigma_bar_v_tilt_2_2]
  [sigma_bar_v_tilt_vec] -> choose ksi_est_err 25/1(x)
  cal theta_sigma_bar_v_tilt agent 3/2(theta_sigma_bar_v_tilt_2_3) -> [theta_sigma_bar_v_tilt_2_3]
  Constant110/1 -> Mux23/2
  [sigma_bar_v_tilt_squ_2_3] -> cal theta_sigma_bar_v_tilt agent 3/3(sigma_bar_v_tilt_squ_2_3)
  [sigma_bar_v_tilt_vec] -> choose ksi_est_err 26/1(x)
  choose ksi_est_err 25/1(y) -> cal abs 25/1(x)
  Mux23/1 -> Interpreted MATLAB Function24/1
  choose ksi_est_err 26/1(y) -> cal abs 26/1(x)
  Constant109/1 -> Mux24/3
  cal abs 25/1(y) -> Mux24/1
  Interpreted MATLAB Function24/1 -> trans to column24/1(x)
  Constant107/1 -> Mux24/2
  Mux24/1 -> Interpreted MATLAB Function25/1
  cal theta_sigma_bar_v_tilt agent 3/1(theta_sigma_bar_v_tilt_1_3) -> [theta_sigma_bar_v_tilt_1_3]
  Constant111/1 -> Mux23/3
  Constant108/1 -> cal theta_sigma_bar_v_tilt agent 3/1(alfa_theta)
  trans to column24/1(y) -> [sigma_bar_v_tilt_squ_2_3], Display54/1
  [sigma_bar_v_tilt_squ_1_3] -> cal theta_sigma_bar_v_tilt agent 3/2(sigma_bar_v_tilt_squ_1_3)
  trans to column25/1(y) -> [sigma_bar_v_tilt_squ_1_3], Display55/1
  Interpreted MATLAB Function25/1 -> trans to column25/1(x)
  [sigma_bar_v_tilt_vec] -> cal theta_sigma_bar_v_tilt agent 3/4(sigma_bar_v_tilt_vec)
  cal abs 26/1(y) -> Mux23/1
  cal abs 28/1(y) -> Mux25/1
  trans to column27/1(y) -> [sigma_bar_v_tilt_squ_1_4], Display57/1
  Interpreted MATLAB Function27/1 -> trans to column27/1(x)
  Constant113/1 -> cal theta_sigma_bar_v_tilt agent 4/1(alfa_theta)
  [sigma_bar_v_tilt_squ_1_4] -> cal theta_sigma_bar_v_tilt agent 4/2(sigma_bar_v_tilt_squ_1_4)
  Constant116/1 -> Mux25/3
  trans to column26/1(y) -> [sigma_bar_v_tilt_squ_2_4], Display56/1
  Constant112/1 -> Mux26/2
  Mux26/1 -> Interpreted MATLAB Function27/1
  [sigma_bar_v_tilt_vec] -> cal theta_sigma_bar_v_tilt agent 4/4(sigma_bar_v_tilt_vec)
  Constant114/1 -> Mux26/3
  cal abs 27/1(y) -> Mux26/1
  cal theta_sigma_bar_v_tilt agent 4/1(theta_sigma_bar_v_tilt_1_4) -> [theta_sigma_bar_v_tilt_1_4]
  Constant115/1 -> Mux25/2
  choose ksi_est_err 27/1(y) -> cal abs 27/1(x)
  choose ksi_est_err 28/1(y) -> cal abs 28/1(x)
  Interpreted MATLAB Function26/1 -> trans to column26/1(x)
  cal theta_sigma_bar_v_tilt agent 4/2(theta_sigma_bar_v_tilt_2_4) -> [theta_sigma_bar_v_tilt_2_4]
  [sigma_bar_v_tilt_vec] -> choose ksi_est_err 28/1(x)
  [sigma_bar_v_tilt_squ_2_4] -> cal theta_sigma_bar_v_tilt agent 4/3(sigma_bar_v_tilt_squ_2_4)
  [sigma_bar_v_tilt_vec] -> choose ksi_est_err 27/1(x)
  Mux25/1 -> Interpreted MATLAB Function26/1
  [sigma_bar_v_tilt_squ_2_5] -> cal theta_sigma_bar_v_tilt agent 5/3(sigma_bar_v_tilt_squ_2_5)
  choose ksi_est_err 29/1(y) -> cal abs 29/1(x)
  Interpreted MATLAB Function28/1 -> trans to column28/1(x)
  choose ksi_est_err 30/1(y) -> cal abs 30/1(x)
  Constant120/1 -> Mux27/2
  cal theta_sigma_bar_v_tilt agent 5/2(theta_sigma_bar_v_tilt_2_5) -> [theta_sigma_bar_v_tilt_2_5]
  [sigma_bar_v_tilt_vec] -> choose ksi_est_err 29/1(x)
  cal theta_sigma_bar_v_tilt agent 5/1(theta_sigma_bar_v_tilt_1_5) -> [theta_sigma_bar_v_tilt_1_5]
  [sigma_bar_v_tilt_vec] -> choose ksi_est_err 30/1(x)
  Constant119/1 -> Mux28/3
  trans to column28/1(y) -> [sigma_bar_v_tilt_squ_2_5], Display58/1
  Mux28/1 -> Interpreted MATLAB Function29/1
  Constant117/1 -> Mux28/2
  cal abs 29/1(y) -> Mux28/1
  [sigma_bar_v_tilt_squ_1_5] -> cal theta_sigma_bar_v_tilt agent 5/2(sigma_bar_v_tilt_squ_1_5)
  Mux27/1 -> Interpreted MATLAB Function28/1
  Constant121/1 -> Mux27/3
  Interpreted MATLAB Function29/1 -> trans to column29/1(x)
  [sigma_bar_v_tilt_vec] -> cal theta_sigma_bar_v_tilt agent 5/4(sigma_bar_v_tilt_vec)
  Constant118/1 -> cal theta_sigma_bar_v_tilt agent 5/1(alfa_theta)
  trans to column29/1(y) -> [sigma_bar_v_tilt_squ_1_5], Display59/1
  cal abs 30/1(y) -> Mux27/1
  combine theta_sigma_bar_v_tilt/1(theta_sigma_bar_v_tilt_1_vec) -> [theta_sigma_bar_v_tilt_1_vec]
  [theta_sigma_bar_v_tilt_2_1] -> combine theta_sigma_bar_v_tilt/6(theta_sigma_bar_v_tilt_2_1)
  [theta_sigma_bar_v_tilt_1_4] -> combine theta_sigma_bar_v_tilt/4(theta_sigma_bar_v_tilt_1_4)
  [theta_sigma_bar_v_tilt_2_2] -> combine theta_sigma_bar_v_tilt/7(theta_sigma_bar_v_tilt_2_2)
  [theta_sigma_bar_v_tilt_1_2] -> combine theta_sigma_bar_v_tilt/2(theta_sigma_bar_v_tilt_1_2)
  [theta_sigma_bar_v_tilt_2_5] -> combine theta_sigma_bar_v_tilt/10(theta_sigma_bar_v_tilt_2_5)
  [theta_sigma_bar_v_tilt_2_4] -> combine theta_sigma_bar_v_tilt/9(theta_sigma_bar_v_tilt_2_4)
  combine theta_sigma_bar_v_tilt/2(theta_sigma_bar_v_tilt_2_vec) -> [theta_sigma_bar_v_tilt_2_vec]
  [theta_sigma_bar_v_tilt_1_1] -> combine theta_sigma_bar_v_tilt/1(theta_sigma_bar_v_tilt_1_1)
  [theta_sigma_bar_v_tilt_2_3] -> combine theta_sigma_bar_v_tilt/8(theta_sigma_bar_v_tilt_2_3)
  [theta_sigma_bar_v_tilt_1_5] -> combine theta_sigma_bar_v_tilt/5(theta_sigma_bar_v_tilt_1_5)
  [theta_sigma_bar_v_tilt_1_3] -> combine theta_sigma_bar_v_tilt/3(theta_sigma_bar_v_tilt_1_3)
  Constant122/1 -> cal sigma_bar_v_hat agent 1/1(c1v)
  Constant123/1 -> cal sigma_bar_v_hat agent 1/2(c2v)
  [theta_sigma_bar_v_tilt_1_vec] -> cal sigma_bar_v_hat agent 1/3(theta_sigma_bar_v_tilt_1_vec)
  [theta_sigma_bar_v_tilt_2_vec] -> cal sigma_bar_v_hat agent 1/4(theta_sigma_bar_v_tilt_2_vec)
  [d_sigma_bar_v_vec] -> cal sigma_bar_v_hat agent 1/5(d_sigma_bar_v_vec)
  cal sigma_bar_v_hat agent 1/1(d_sigma_bar_v_hat_1) -> sigma_bar_v_hat Integrator 1/1
  [theta_sigma_bar_v_tilt_2_vec] -> cal sigma_bar_v_hat agent 2/4(theta_sigma_bar_v_tilt_2_vec)
  Constant125/1 -> cal sigma_bar_v_hat agent 2/2(c2v)
  cal sigma_bar_v_hat agent 2/1(d_sigma_bar_v_hat_2) -> sigma_bar_v_hat Integrator 2/1
  [d_sigma_bar_v_vec] -> cal sigma_bar_v_hat agent 2/5(d_sigma_bar_v_vec)
  [theta_sigma_bar_v_tilt_1_vec] -> cal sigma_bar_v_hat agent 2/3(theta_sigma_bar_v_tilt_1_vec)
  Constant124/1 -> cal sigma_bar_v_hat agent 2/1(c1v)
  Constant126/1 -> cal sigma_bar_v_hat agent 3/1(c1v)
  [theta_sigma_bar_v_tilt_2_vec] -> cal sigma_bar_v_hat agent 3/4(theta_sigma_bar_v_tilt_2_vec)
  cal sigma_bar_v_hat agent 3/1(d_sigma_bar_v_hat_3) -> sigma_bar_v_hat Integrator 3/1
  [d_sigma_bar_v_vec] -> cal sigma_bar_v_hat agent 3/5(d_sigma_bar_v_vec)
  Constant127/1 -> cal sigma_bar_v_hat agent 3/2(c2v)
  [theta_sigma_bar_v_tilt_1_vec] -> cal sigma_bar_v_hat agent 3/3(theta_sigma_bar_v_tilt_1_vec)
  [d_sigma_bar_v_vec] -> cal sigma_bar_v_hat agent 4/5(d_sigma_bar_v_vec)
  [theta_sigma_bar_v_tilt_1_vec] -> cal sigma_bar_v_hat agent 4/3(theta_sigma_bar_v_tilt_1_vec)
  Constant139/1 -> cal sigma_bar_v_hat agent 4/2(c2v)
  cal sigma_bar_v_hat agent 4/1(d_sigma_bar_v_hat_4) -> sigma_bar_v_hat Integrator 4/1
  [theta_sigma_bar_v_tilt_2_vec] -> cal sigma_bar_v_hat agent 4/4(theta_sigma_bar_v_tilt_2_vec)
  Constant128/1 -> cal sigma_bar_v_hat agent 4/1(c1v)
  [sigma_bar_v_hat_5] -> combine sigma_bar_v_hat/5(sigma_bar_v_hat_5)
  [sigma_bar_v_hat_4] -> combine sigma_bar_v_hat/4(sigma_bar_v_hat_4)
  [sigma_bar_v_hat_3] -> combine sigma_bar_v_hat/3(sigma_bar_v_hat_3)
  combine sigma_bar_v_hat/1(sigma_bar_v_hat_vec) -> [sigma_bar_v_hat_vec]
  cal combine sigma_bar_v_tilt/1(sigma_bar_v_tilt_vec) -> [sigma_bar_v_tilt_vec]
  [sigma_bar_v_vec] -> cal combine sigma_bar_v_tilt/1(sigma_bar_v_vec)
  [sigma_bar_v_hat_vec] -> cal combine sigma_bar_v_tilt/2(sigma_bar_v_hat_vec)
  [sigma_bar_v_hat_2] -> combine sigma_bar_v_hat/2(sigma_bar_v_hat_2)
  [sigma_bar_v_hat_1] -> combine sigma_bar_v_hat/1(sigma_bar_v_hat_1)
  sigma_bar_v_hat Integrator 1/1 -> [sigma_bar_v_hat_1]
  sigma_bar_v_hat Integrator 2/1 -> [sigma_bar_v_hat_2]
  sigma_bar_v_hat Integrator 3/1 -> [sigma_bar_v_hat_3]
  sigma_bar_v_hat Integrator 4/1 -> [sigma_bar_v_hat_4]
  sigma_bar_v_hat Integrator 5/1 -> [sigma_bar_v_hat_5]
  [d_sigma_bar_v_vec] -> cal sigma_bar_v_hat agent 5/5(d_sigma_bar_v_vec)
  [theta_sigma_bar_v_tilt_2_vec] -> cal sigma_bar_v_hat agent 5/4(theta_sigma_bar_v_tilt_2_vec)
  cal sigma_bar_v_hat agent 5/1(d_sigma_bar_v_hat_5) -> sigma_bar_v_hat Integrator 5/1
  [theta_sigma_bar_v_tilt_1_vec] -> cal sigma_bar_v_hat agent 5/3(theta_sigma_bar_v_tilt_1_vec)
  Constant141/1 -> cal sigma_bar_v_hat agent 5/2(c2v)
  Constant140/1 -> cal sigma_bar_v_hat agent 5/1(c1v)
  Constant142/1 -> cal dp_hat agent 1/1(c3v)
  [d_sigma_bar_v_vec] -> cal dp_hat agent 1/2(d_sigma_bar_v_vec)
  [sigma_bar_v_hat_vec] -> cal dp_hat agent 1/3(sigma_bar_v_hat_vec)
  cal dp_hat agent 1/1(dp_hat_1) -> [dp_hat_1]
  cal dp_hat agent 2/1(dp_hat_2) -> [dp_hat_2]
  [d_sigma_bar_v_vec] -> cal dp_hat agent 2/2(d_sigma_bar_v_vec)
  Constant143/1 -> cal dp_hat agent 2/1(c3v)
  [sigma_bar_v_hat_vec] -> cal dp_hat agent 2/3(sigma_bar_v_hat_vec)
  [sigma_bar_v_hat_vec] -> cal dp_hat agent 3/3(sigma_bar_v_hat_vec)
  Constant144/1 -> cal dp_hat agent 3/1(c3v)
  [d_sigma_bar_v_vec] -> cal dp_hat agent 3/2(d_sigma_bar_v_vec)
  cal dp_hat agent 3/1(dp_hat_3) -> [dp_hat_3]
  cal dp_hat agent 4/1(dp_hat_4) -> [dp_hat_4]
  [d_sigma_bar_v_vec] -> cal dp_hat agent 4/2(d_sigma_bar_v_vec)
  Constant145/1 -> cal dp_hat agent 4/1(c3v)
  [sigma_bar_v_hat_vec] -> cal dp_hat agent 4/3(sigma_bar_v_hat_vec)
  cal dp_hat agent 5/1(dp_hat_5) -> [dp_hat_5]
  [sigma_bar_v_hat_vec] -> cal dp_hat agent 5/3(sigma_bar_v_hat_vec)
  Constant146/1 -> cal dp_hat agent 5/1(c3v)
  [d_sigma_bar_v_vec] -> cal dp_hat agent 5/2(d_sigma_bar_v_vec)
  combine dp_hat/1(dp_hat_vec) -> [dp_hat_vec]
  [dp_hat_1] -> combine dp_hat/1(dp_hat_1)
  [dp_hat_4] -> combine dp_hat/4(dp_hat_4)
  [dp_hat_3] -> combine dp_hat/3(dp_hat_3)
  [dp_hat_5] -> combine dp_hat/5(dp_hat_5)
  [dp_hat_2] -> combine dp_hat/2(dp_hat_2)
  cal ui agent 1/1(ui_1) -> [ui_1]
  [ui_5] -> combine ui/5(ui_5)
  [ui_2] -> combine ui/2(ui_2)
  [ui_1] -> combine ui/1(ui_1)
  [ui_4] -> combine ui/4(ui_4)
  [ui_3] -> combine ui/3(ui_3)
  combine ui/1(ui_vec) -> [ui]
  Phi_sec_sigma_i agent 1/1(Phi_sec_sigma_1) -> [Phi_sec_sigma_1]
  Phi_sec_sigma_i agent 5/1(Phi_sec_sigma_5) -> [Phi_sec_sigma_5]
  combine Phi_sec_sigma_i/1(Phi_sec_sigma_vec) -> Memory/1
  [Phi_sec_sigma_5] -> combine Phi_sec_sigma_i/5(Phi_sec_sigma_5)
  [Phi_sec_sigma_1] -> combine Phi_sec_sigma_i/1(Phi_sec_sigma_1)
  [sigmai_vec] -> Phi_sec_sigma_i agent 2/1(sigma_i_vec)
  [Phi_sec_sigma_4] -> combine Phi_sec_sigma_i/4(Phi_sec_sigma_4)
  Phi_sec_sigma_i agent 4/1(Phi_sec_sigma_4) -> [Phi_sec_sigma_4]
  Phi_sec_sigma_i agent 3/1(Phi_sec_sigma_3) -> [Phi_sec_sigma_3]
  [sigmai_vec] -> Phi_sec_sigma_i agent 5/1(sigma_i_vec)
  Phi_sec_sigma_i agent 2/1(Phi_sec_sigma_2) -> [Phi_sec_sigma_2]
  [sigmai_vec] -> Phi_sec_sigma_i agent 1/1(sigma_i_vec)
  [Phi_sec_sigma_2] -> combine Phi_sec_sigma_i/2(Phi_sec_sigma_2)
  [Phi_sec_sigma_3] -> combine Phi_sec_sigma_i/3(Phi_sec_sigma_3)
  [sigmai_vec] -> Phi_sec_sigma_i agent 3/1(sigma_i_vec)
  Memory/1 -> [Phi_sec_sigma_vec]
  [sigmai_vec] -> Phi_sec_sigma_i agent 4/1(sigma_i_vec)
  Constant2/1 -> update betai agent 1/3(Mii)
  [u0] -> update betai agent 3/5(u0)
  [tsim] -> update betai agent 4/4(tsim)
  [rho_hat_vec] -> update betai agent 2/6(rho_hat_vec)
  Constant4/1 -> update betai agent 2/2(Wij)
  Constant13/1 -> update betai agent 5/3(Mii)
  Constant3/1 -> update betai agent 2/1(eps0)
  [u0] -> update betai agent 2/5(u0)
  beta_hat Integrator 1/1 -> [beta_hat_1]
  beta_hat Integrator 2/1 -> [beta_hat_2]
  Constant12/1 -> update betai agent 5/2(Wij)
  [u0] -> update betai agent 5/5(u0)
  [rho_hat_vec] -> update betai agent 1/6(rho_hat_vec)
  Constant14/1 -> update betai agent 5/1(eps0)
  [tsim] -> update betai agent 2/4(tsim)
  combine betai/1(beta_hat_vec) -> Memory4/1
  [beta_hat_5] -> combine betai/5(beta_hat_5)
  [beta_hat_3] -> combine betai/3(beta_hat_3)
  [beta_hat_4] -> combine betai/4(beta_hat_4)
  [beta_hat_2] -> combine betai/2(beta_hat_2)
  Memory4/1 -> [beta_hat_vec]
  beta_hat Integrator 5/1 -> [beta_hat_5]
  beta_hat Integrator 4/1 -> [beta_hat_4]
  update betai agent 5/1(d_beta_hat_5) -> beta_hat Integrator 5/1
  [beta_hat_1] -> combine betai/1(beta_hat_1)
  Constant9/1 -> update betai agent 4/1(eps0)
  Constant10/1 -> update betai agent 4/2(Wij)
  [tsim] -> update betai agent 3/4(tsim)
  Constant11/1 -> update betai agent 4/3(Mii)
  [rho_hat_vec] -> update betai agent 4/6(rho_hat_vec)
  Constant8/1 -> update betai agent 3/3(Mii)
  beta_hat Integrator 3/1 -> [beta_hat_3]
  Constant7/1 -> update betai agent 3/2(Wij)
  Constant1/1 -> update betai agent 1/2(Wij)
  [tsim] -> update betai agent 1/4(tsim)
  update betai agent 2/1(d_beta_hat_2) -> beta_hat Integrator 2/1
  [u0] -> update betai agent 1/5(u0)
  [tsim] -> update betai agent 5/4(tsim)
  update betai agent 3/1(d_beta_hat_3) -> beta_hat Integrator 3/1
  update betai agent 1/1(d_beta_hat_1) -> beta_hat Integrator 1/1
  [u0] -> update betai agent 4/5(u0)
  Constant/1 -> update betai agent 1/1(eps0)
  Constant6/1 -> update betai agent 3/1(eps0)
  [rho_hat_vec] -> update betai agent 3/6(rho_hat_vec)
  Constant5/1 -> update betai agent 2/3(Mii)
  [rho_hat_vec] -> update betai agent 5/6(rho_hat_vec)
  update betai agent 4/1(d_beta_hat_4) -> beta_hat Integrator 4/1
  update sigmai agent 3/1(d_sigmai_3) -> sigmai Integrator 3/1
  [beta_hat_vec] -> update sigmai agent 3/8(beta_hat_vec)
  [sigmai_4] -> combine betai1/4(sigmai_4)
  Constant19/1 -> update sigmai agent 1/5(Mii)
  Constant33/1 -> update sigmai agent 4/4(Wij)
  [Phi_sec_sigma_vec] -> update sigmai agent 1/10(Phi_sec_sigma_vec)
  Constant31/1 -> update sigmai agent 4/2(lam0)
  Memory5/1 -> [sigmai_vec]
  [Phi_sec_sigma_vec] -> update sigmai agent 5/10(Phi_sec_sigma_vec)
  Constant39/1 -> update sigmai agent 5/5(Mii)
  sigmai Integrator 5/1 -> [sigmai_5]
  Constant37/1 -> update sigmai agent 5/3(eps0)
  Constant38/1 -> update sigmai agent 5/4(Wij)
  update sigmai agent 5/1(d_sigmai_5) -> sigmai Integrator 5/1
  Constant26/1 -> update sigmai agent 3/2(lam0)
  [beta_hat_vec] -> update sigmai agent 5/8(beta_hat_vec)
  [u0] -> update sigmai agent 5/7(u0)
  [u0] -> update sigmai agent 4/7(u0)
  Constant32/1 -> update sigmai agent 4/3(eps0)
  sigmai Integrator 4/1 -> [sigmai_4]
  combine betai1/1(sigmai_vec) -> Memory5/1
  [tsim] -> update sigmai agent 4/6(tsim)
  [Phi_sec_sigma_vec] -> update sigmai agent 3/10(Phi_sec_sigma_vec)
  Constant28/1 -> update sigmai agent 3/4(Wij)
  [tsim] -> update sigmai agent 3/6(tsim)
  [rho_hat_vec] -> update sigmai agent 4/9(rho_hat_vec)
  [u0] -> update sigmai agent 2/7(u0)
  Constant34/1 -> update sigmai agent 4/5(Mii)
  [sigmai_3] -> combine betai1/3(sigmai_3)
  Constant22/1 -> update sigmai agent 2/3(eps0)
  [Phi_sec_sigma_vec] -> update sigmai agent 2/10(Phi_sec_sigma_vec)
  sigmai Integrator 1/1 -> [sigmai_1]
  update sigmai agent 2/1(d_sigmai_2) -> sigmai Integrator 2/1
  [tsim] -> update sigmai agent 2/6(tsim)
  [sigmai_5] -> combine betai1/5(sigmai_5)
  sigmai Integrator 3/1 -> [sigmai_3]
  [rho_hat_vec] -> update sigmai agent 2/9(rho_hat_vec)
  Constant24/1 -> update sigmai agent 2/5(Mii)
  Constant27/1 -> update sigmai agent 3/3(eps0)
  [beta_hat_vec] -> update sigmai agent 2/8(beta_hat_vec)
  Constant23/1 -> update sigmai agent 2/4(Wij)
  [u0] -> update sigmai agent 1/7(u0)
  Constant18/1 -> update sigmai agent 1/4(Wij)
  Constant17/1 -> update sigmai agent 1/3(eps0)
  [sigmai_2] -> combine betai1/2(sigmai_2)
  [tsim] -> update sigmai agent 1/6(tsim)
  [rho_hat_vec] -> update sigmai agent 3/9(rho_hat_vec)
  [rho_hat_vec] -> update sigmai agent 1/9(rho_hat_vec)
  Constant21/1 -> update sigmai agent 2/2(lam0)
  Constant15/1 -> update sigmai agent 1/1(kai0)
  Constant16/1 -> update sigmai agent 1/2(lam0)
  Constant35/1 -> update sigmai agent 5/1(kai0)
  Constant36/1 -> update sigmai agent 5/2(lam0)
  [beta_hat_vec] -> update sigmai agent 1/8(beta_hat_vec)
  [tsim] -> update sigmai agent 5/6(tsim)
  [beta_hat_vec] -> update sigmai agent 4/8(beta_hat_vec)
  sigmai Integrator 2/1 -> [sigmai_2]
  Constant20/1 -> update sigmai agent 2/1(kai0)
  [u0] -> update sigmai agent 3/7(u0)
  Constant29/1 -> update sigmai agent 3/5(Mii)
  Constant30/1 -> update sigmai agent 4/1(kai0)
  [Phi_sec_sigma_vec] -> update sigmai agent 4/10(Phi_sec_sigma_vec)
  [sigmai_1] -> combine betai1/1(sigmai_1)
  Constant25/1 -> update sigmai agent 3/1(kai0)
  update sigmai agent 1/1(d_sigmai_1) -> sigmai Integrator 1/1
  update sigmai agent 4/1(d_sigmai_4) -> sigmai Integrator 4/1
  [rho_hat_vec] -> update sigmai agent 5/9(rho_hat_vec)
  choose rho_hat agent 3/1(y) -> Demux41/1
  rho_hat agent 5/1(rho_hat_5) -> [rho_hat_5]
  Demux43/2 -> Mux8/2
  Demux45/1 -> Mux10/2
  Demux45/2 -> Mux11/2
  Demux43/3 -> Mux9/2
  Demux33/1 -> Mux10/1
  choose rho_hat agent 5/1(y) -> Demux45/1
  Demux33/3 -> Mux12/1
  [u0] -> Demux44/1
  Mux4/1 -> u0 vs rho_hat agent 3/1
  Mux12/1 -> u0 vs rho_hat agent 5/3
  Mux11/1 -> u0 vs rho_hat agent 5/2
  Demux41/1 -> Mux4/2
  [rho_hat_2] -> combine rho_hat/2(rho_hat_2)
  [rho_hat_vec] -> cal rho_err_vec/2(rho_hat_vec)
  [rho_hat_vec] -> choose rho_hat agent 5/1(x)
  Demux38/3 -> Mux135/2
  Demux44/2 -> Mux8/1
  Constant40/1 -> rho_hat agent 1/1(lam0)
  Demux41/2 -> Mux5/2
  Mux7/1 -> u0 vs rho_hat agent 4/1
  Demux44/1 -> Mux7/1
  Mux9/1 -> u0 vs rho_hat agent 4/3
  Memory6/1 -> [rho_hat_vec]
  Mux8/1 -> u0 vs rho_hat agent 4/2
  Mux5/1 -> u0 vs rho_hat agent 3/2
  Constant41/1 -> rho_hat agent 2/1(lam0)
  Demux43/1 -> Mux7/2
  [rho_hat_vec] -> choose rho_hat agent 3/1(x)
  [u0] -> Demux42/1
  choose rho_hat agent 4/1(y) -> Demux43/1
  Demux42/2 -> Mux5/1
  [u0] -> Demux40/1
  Demux42/3 -> Mux6/1
  Demux40/3 -> Mux3/1
  Demux39/1 -> Mux1/2
  [rho_hat_vec] -> choose rho_hat agent 2/1(x)
  Mux3/1 -> u0 vs rho_hat agent 2/3
  Demux39/3 -> Mux3/2
  Demux94/3 -> Mux135/1
  Demux38/1 -> Mux133/2
  [rho_hat_5] -> combine rho_hat/5(rho_hat_5)
  rho_hat agent 2/1(rho_hat_2) -> [rho_hat_2]
  [rho_hat_1] -> combine rho_hat/1(rho_hat_1)
  rho_hat agent 3/1(rho_hat_3) -> [rho_hat_3]
  Mux135/1 -> u0 vs rho_hat agent 1/3
  choose rho_hat agent 2/1(y) -> Demux39/1
  Mux134/1 -> u0 vs rho_hat agent 1/2
  Constant44/1 -> rho_hat agent 5/1(lam0)
  Mux2/1 -> u0 vs rho_hat agent 2/2
  [sigmai_vec] -> rho_hat agent 4/2(sigmai_vec)
  Constant43/1 -> rho_hat agent 4/1(lam0)
  Demux41/3 -> Mux6/2
  [sigmai_vec] -> rho_hat agent 1/2(sigmai_vec)
  combine rho_hat/1(rho_hat_vec) -> Memory6/1
  Demux44/3 -> Mux9/1
  Demux94/2 -> Mux134/1
  Mux133/1 -> u0 vs rho_hat agent 1/1
  [rho_hat_vec] -> choose rho_hat agent 4/1(x)
  Constant42/1 -> rho_hat agent 3/1(lam0)
  Demux40/2 -> Mux2/1
  [u0] -> Demux94/1
  Demux39/2 -> Mux2/2
  rho_hat agent 4/1(rho_hat_4) -> [rho_hat_4]
  [rho_hat_vec] -> choose rho_hat agent 1/1(x)
  [rho_hat_4] -> combine rho_hat/4(rho_hat_4)
  [sigmai_vec] -> rho_hat agent 5/2(sigmai_vec)
  Demux33/2 -> Mux11/1
  Demux94/1 -> Mux133/1
  [rho_hat_3] -> combine rho_hat/3(rho_hat_3)
  [u0] -> Demux33/1
  Demux45/3 -> Mux12/2
  cal rho_err_vec/1(rho_err_vec) -> [rho_err_vec]
  Mux6/1 -> u0 vs rho_hat agent 3/3
  [u0] -> cal rho_err_vec/1(u0)
  [sigmai_vec] -> rho_hat agent 3/2(sigmai_vec)
  rho_hat agent 1/1(rho_hat_1) -> [rho_hat_1]
  choose rho_hat agent 1/1(y) -> Demux38/1
  Mux10/1 -> u0 vs rho_hat agent 5/1
  [sigmai_vec] -> rho_hat agent 2/2(sigmai_vec)
  Demux42/1 -> Mux4/1
  Mux1/1 -> u0 vs rho_hat agent 2/1
  Demux40/1 -> Mux1/1
  Demux38/2 -> Mux134/2
  Constant45/1 -> update dpsy psy agent 1/1(Wij)
  Constant46/1 -> update dpsy psy agent 1/2(Mii)
  [ksi_i_vec] -> update dpsy psy agent 1/5(ksi_i_vec)
  [eta_i_vec] -> update dpsy psy agent 1/6(eta_i_vec)
  [ksi_d_est_vec] -> update dpsy psy agent 1/7(ksi_d_est_vec)
  [eta_d_est_vec] -> update dpsy psy agent 1/8(eta_d_est_vec)
  update dpsy psy agent 1/1(d_2_psy_1) -> d_psy Integrator 1/1
  d_psy Integrator 1/1 -> [d_psy_1], psy Integrator 1/1
  psy Integrator 1/1 -> [psy_1]
  [d_psy_4] -> combine d_psy/4(d_psy_4)
  [d_psy_1] -> combine d_psy/1(d_psy_1)
  [d_psy_2] -> combine d_psy/2(d_psy_2)
  [d_psy_3] -> combine d_psy/3(d_psy_3)
  combine d_psy/1(d_psy_vec) -> Memory3/1
  [d_psy_5] -> combine d_psy/5(d_psy_5)
  [psy_2] -> combine psy/2(psy_2)
  [psy_3] -> combine psy/3(psy_3)
  [psy_5] -> combine psy/5(psy_5)
  [psy_4] -> combine psy/4(psy_4)
  [psy_1] -> combine psy/1(psy_1)
  combine psy/1(psy_vec) -> Memory7/1
  [d_psy_vec] -> cal eta_d_est ksi_d_est/1(d_psy_vec)
  [psy_vec] -> cal eta_d_est ksi_d_est/2(psy_vec)
  [eta_i_vec] -> cal eta_d_est ksi_d_est/3(eta_i_vec)
  [ksi_i_vec] -> cal eta_d_est ksi_d_est/4(ksi_i_vec)
  cal eta_d_est ksi_d_est/1(eta_d_est_vec) -> [eta_d_est_vec]
  cal eta_d_est ksi_d_est/2(ksi_d_est_vec) -> [ksi_d_est_vec]
  Constant61/1 -> cal si agent 1/1(Wij)
  Constant62/1 -> cal si agent 1/2(Mii)
  [ksi0] -> cal si agent 1/4(ksi0)
  [ksi_i_vec] -> cal si agent 1/5(ksi_i_vec)
  [ksi_d_est_vec] -> cal si agent 1/6(ksi_d_est_vec)
  cal si agent 1/1(si_1) -> [si_1]
  [si_2] -> combine si/2(si_2)
  [si_3] -> combine si/3(si_3)
  [si_5] -> combine si/5(si_5)
  [si_4] -> combine si/4(si_4)
  [si_1] -> combine si/1(si_1)
  combine si/1(si_vec) -> [si_vec]
  cal ri agent 1/1(ri_1) -> [ri_1]
  Constant76/1 -> cal ri agent 1/1(Wij)
  Constant77/1 -> cal ri agent 1/2(Mii)
  [eta0] -> cal ri agent 1/4(eta0)
  [eta_i_vec] -> cal ri agent 1/5(eta_i_vec)
  [ri_2] -> combine ri/2(ri_2)
  combine ri/1(ri_vec) -> [ri_vec]
  [ri_1] -> combine ri/1(ri_1)
  [ri_4] -> combine ri/4(ri_4)
  [ri_5] -> combine ri/5(ri_5)
  [ri_3] -> combine ri/3(ri_3)
  Memory3/1 -> [d_psy_vec]
  Memory7/1 -> [psy_vec]
  Constant86/1 -> cal ui agent 1/1(c1)
  Constant156/1 -> cal ui agent 1/2(c2)
  Constant87/1 -> cal ui agent 1/3(sat_sr_up)
  Constant88/1 -> cal ui agent 1/4(sat_sr_low)
  [rho_hat_vec] -> cal ui agent 1/5(rho_hat_vec)
  [dp_hat_vec] -> cal ui agent 1/6(dp_hat_vec)
  [si_vec] -> cal ui agent 1/7(si_vec)
  [ri_vec] -> cal ui agent 1/8(ri_vec)
  Constant91/1 -> cal ui agent 2/3(sat_sr_up)
  [ri_vec] -> cal ui agent 2/8(ri_vec)
  Constant147/1 -> cal ui agent 2/4(sat_sr_low)
  Constant89/1 -> cal ui agent 2/2(c2)
  [si_vec] -> cal ui agent 2/7(si_vec)
  Constant90/1 -> cal ui agent 2/1(c1)
  [rho_hat_vec] -> cal ui agent 2/5(rho_hat_vec)
  [dp_hat_vec] -> cal ui agent 2/6(dp_hat_vec)
  cal ui agent 2/1(ui_2) -> [ui_2]
  [ri_vec] -> cal ui agent 3/8(ri_vec)
  Constant151/1 -> cal ui agent 3/3(sat_sr_up)
  Constant148/1 -> cal ui agent 3/4(sat_sr_low)
  Constant149/1 -> cal ui agent 3/2(c2)
  [dp_hat_vec] -> cal ui agent 3/6(dp_hat_vec)
  Constant150/1 -> cal ui agent 3/1(c1)
  [rho_hat_vec] -> cal ui agent 3/5(rho_hat_vec)
  [si_vec] -> cal ui agent 3/7(si_vec)
  cal ui agent 3/1(ui_3) -> [ui_3]
  Constant154/1 -> cal ui agent 4/1(c1)
  [rho_hat_vec] -> cal ui agent 4/5(rho_hat_vec)
  Constant153/1 -> cal ui agent 4/2(c2)
  Constant152/1 -> cal ui agent 4/4(sat_sr_low)
  cal ui agent 4/1(ui_4) -> [ui_4]
  Constant155/1 -> cal ui agent 4/3(sat_sr_up)
  [dp_hat_vec] -> cal ui agent 4/6(dp_hat_vec)
  [ri_vec] -> cal ui agent 4/8(ri_vec)
  [si_vec] -> cal ui agent 4/7(si_vec)
  [si_vec] -> cal ui agent 5/7(si_vec)
  [dp_hat_vec] -> cal ui agent 5/6(dp_hat_vec)
  [rho_hat_vec] -> cal ui agent 5/5(rho_hat_vec)
  Constant157/1 -> cal ui agent 5/4(sat_sr_low)
  Constant159/1 -> cal ui agent 5/1(c1)
  [ri_vec] -> cal ui agent 5/8(ri_vec)
  cal ui agent 5/1(ui_5) -> [ui_5]
  Constant160/1 -> cal ui agent 5/3(sat_sr_up)
  Constant158/1 -> cal ui agent 5/2(c2)
  [eta_d_est_vec] -> cal ri agent 1/6(eta_d_est_vec)
  Constant222/1 -> set desire formation configuration/8(Z2)
  leader ksi0 Integrator/1 -> [ksi0]
  leader control input/1(u0) -> [u0]
  Demux1/1 -> ksi_0/1
  Constant238/1 -> set desire formation configuration/13(T1)
  Constant226/1 -> set desire formation configuration/9(Z3)
  Constant165/1 -> process velocity/1(T0)
  desire formation position and velocity/1(pos_i_des) -> [pos_i_des]
  Constant176/1 -> leader control input/6(Rx2)
  Constant231/1 -> set desire formation configuration/11(kai_1_t)
  [delta_ksi_vec] -> desire formation position and velocity/3(delta_ksi_vec)
  Constant181/1 -> process velocity/4(PZ0)
  Constant173/1 -> leader control input/3(T2)
  set desire formation configuration/2(delta_eta_vec) -> [delta_eta_vec]
  Constant225/1 -> set desire formation configuration/10(theta0)
  [V_init_out] -> leader eta0 Integrator/3
  process velocity/1(V_init_out) -> [V_init_out]
  Demux1/3 -> ksi_0/3
  Constant235/1 -> set desire formation configuration/12(kai_3_t)
  desire formation position and velocity/2(vel_i_des) -> [vel_i_des]
  set desire formation configuration/3(d_delta_eta_vec) -> [d_delta_eta_vec]
  Constant166/1 -> process velocity/10(Rz2)
  leader eta0 Integrator/1 -> [eta0], leader ksi0 Integrator/1
  Clock/1 -> [tsim]
  [tsim] -> process velocity/11(t)
  Constant221/1 -> set desire formation configuration/7(Z1)
  Constant175/1 -> leader control input/5(R1)
  Demux22/2 -> eta_0/2
  Constant169/1 -> set desire formation configuration/1(X1)
  Constant178/1 -> leader control input/8(Rz2)
  Constant239/1 -> set desire formation configuration/14(T12)
  Constant180/1 -> process velocity/2(T1)
  Constant172/1 -> set desire formation configuration/5(Y2)
  [u0] -> leader eta0 Integrator/1
  Constant174/1 -> leader control input/4(R0)
  Constant177/1 -> leader control input/7(Ry2)
  [delta_eta_vec] -> desire formation position and velocity/4(delta_eta_vec)
  Constant182/1 -> process velocity/5(PZ1)
  Demux22/3 -> eta_0/3
  Constant167/1 -> process velocity/9(Ry2)
  Demux1/2 -> ksi_0/2
  Constant179/1 -> process velocity/3(T2)
  Constant162/1 -> leader control input/2(T1)
  Constant168/1 -> process velocity/8(Rx2)
  [eta0] -> Demux22/1
  [ksi0] -> desire formation position and velocity/1(ksi0)
  Constant170/1 -> set desire formation configuration/2(X2)
  [tsim] -> set desire formation configuration/15(t)
  Constant234/1 -> set desire formation configuration/3(X3)
  Step/1 -> leader eta0 Integrator/2
  [ksi0] -> Demux1/1
  Constant163/1 -> process velocity/6(R0)
  [tsim] -> leader control input/1(t)
  Constant171/1 -> set desire formation configuration/4(Y1)
  set desire formation configuration/1(delta_ksi_vec) -> [delta_ksi_vec]
  [eta0] -> desire formation position and velocity/2(eta0)
  Constant229/1 -> set desire formation configuration/6(Y3)
  Demux22/1 -> eta_0/1
  Constant164/1 -> process velocity/7(R1)
  [sigma_bar_v_vec] -> To Workspace12/1
  [u0] -> To Workspace3/1
  [eta_track_err_vec] -> To Workspace10/1
  [ksi_i_vec] -> To Workspace8/1
  [ksi0] -> To Workspace5/1
  [d_psy_vec] -> To Workspace20/1
  [eta_i_vec] -> To Workspace7/1
  [si_vec] -> To Workspace22/1
  [rho_err_vec] -> To Workspace15/1
  [psy_vec] -> To Workspace16/1
  [beta_hat_vec] -> To Workspace18/1
  [sigma_bar_v_tilt_vec] -> To Workspace13/1
  [sigma_bar_v_hat_vec] -> To Workspace11/1
  [eta0] -> To Workspace4/1
  [dp_vec] -> To Workspace2/1
  [sigmai_vec] -> To Workspace/1
  [dp_tilt_vec] -> To Workspace6/1
  [sigma_v_vec] -> To Workspace19/1
  [rho_hat_vec] -> To Workspace17/1
  [ksi_track_err_vec] -> To Workspace9/1
  [dp_hat_vec] -> To Workspace1/1
  [ui_vec] -> To Workspace14/1
  [ri_vec] -> To Workspace21/1
  [tsim] -> generate translational disturbance agent 3/4(t)
  [dp_1] -> combine translational disturbance/1(dp_1)
  [dp_2] -> combine translational disturbance/2(dp_2)
  [tsim] -> generate translational disturbance agent 5/4(t)
  [tsim] -> generate translational disturbance agent 2/4(t)
  [dp_hat_vec] -> cal disturbance observation error dp_tilt/2(dp_hat_vec)
  generate translational disturbance agent 2/1(dp_2) -> [dp_2]
  generate translational disturbance agent 3/1(dp_3) -> [dp_3]
  Constant244/1 -> generate translational disturbance agent 1/2(dp_ff_t)
  Constant289/1 -> generate translational disturbance agent 3/3(dp_phi_t)
  generate translational disturbance agent 4/1(dp_4) -> [dp_4]
  Constant287/1 -> generate translational disturbance agent 2/2(dp_ff_t)
  Constant292/1 -> generate translational disturbance agent 4/3(dp_phi_t)
  [tsim] -> generate translational disturbance agent 4/4(t)
  generate translational disturbance agent 1/1(dp_1) -> [dp_1]
  Constant294/1 -> generate translational disturbance agent 4/1(dp_aa_t)
  Constant285/1 -> generate translational disturbance agent 1/1(dp_aa_t)
  Constant290/1 -> generate translational disturbance agent 3/2(dp_ff_t)
  Constant243/1 -> generate translational disturbance agent 1/3(dp_phi_t)
  Constant288/1 -> generate translational disturbance agent 2/1(dp_aa_t)
  generate translational disturbance agent 5/1(dp_5) -> [dp_5]
  Constant297/1 -> generate translational disturbance agent 5/1(dp_aa_t)
  [tsim] -> generate translational disturbance agent 1/4(t)
  Constant293/1 -> generate translational disturbance agent 4/2(dp_ff_t)
  Constant286/1 -> generate translational disturbance agent 2/3(dp_phi_t)
  [dp_4] -> combine translational disturbance/4(dp_4)
  cal disturbance observation error dp_tilt/1(dp_tilt_vec) -> [dp_tilt_vec]
  Constant291/1 -> generate translational disturbance agent 3/1(dp_aa_t)
  Constant296/1 -> generate translational disturbance agent 5/2(dp_ff_t)
  [dp_3] -> combine translational disturbance/3(dp_3)
  [dp_vec] -> cal disturbance observation error dp_tilt/1(dp_vec)
  combine translational disturbance/1(dp_vec) -> [dp_vec]
  Constant295/1 -> generate translational disturbance agent 5/3(dp_phi_t)
  [dp_5] -> combine translational disturbance/5(dp_5)
  [delta_ksi_vec] -> update dpsy psy agent 1/3(delta_ksi_vec)
  [delta_eta_vec] -> update dpsy psy agent 1/4(delta_eta_vec)
  [eta_i_vec] -> update dpsy psy agent 2/6(eta_i_vec)
  [ksi_d_est_vec] -> update dpsy psy agent 2/7(ksi_d_est_vec)
  [eta_d_est_vec] -> update dpsy psy agent 2/8(eta_d_est_vec)
  Constant48/1 -> update dpsy psy agent 2/2(Mii)
  d_psy Integrator 2/1 -> [d_psy_2], psy Integrator 2/1
  [delta_ksi_vec] -> update dpsy psy agent 2/3(delta_ksi_vec)
  psy Integrator 2/1 -> [psy_2]
  update dpsy psy agent 2/1(d_2_psy_2) -> d_psy Integrator 2/1
  [delta_eta_vec] -> update dpsy psy agent 2/4(delta_eta_vec)
  Constant47/1 -> update dpsy psy agent 2/1(Wij)
  [ksi_i_vec] -> update dpsy psy agent 2/5(ksi_i_vec)
  psy Integrator 3/1 -> [psy_3]
  [ksi_i_vec] -> update dpsy psy agent 3/5(ksi_i_vec)
  [delta_eta_vec] -> update dpsy psy agent 3/4(delta_eta_vec)
  Constant49/1 -> update dpsy psy agent 3/1(Wij)
  update dpsy psy agent 3/1(d_2_psy_3) -> d_psy Integrator 3/1
  d_psy Integrator 3/1 -> [d_psy_3], psy Integrator 3/1
  [delta_ksi_vec] -> update dpsy psy agent 3/3(delta_ksi_vec)
  [eta_d_est_vec] -> update dpsy psy agent 3/8(eta_d_est_vec)
  [ksi_d_est_vec] -> update dpsy psy agent 3/7(ksi_d_est_vec)
  Constant50/1 -> update dpsy psy agent 3/2(Mii)
  [eta_i_vec] -> update dpsy psy agent 3/6(eta_i_vec)
  [eta_i_vec] -> update dpsy psy agent 4/6(eta_i_vec)
  Constant53/1 -> update dpsy psy agent 4/2(Mii)
  update dpsy psy agent 4/1(d_2_psy_4) -> d_psy Integrator 4/1
  [delta_eta_vec] -> update dpsy psy agent 4/4(delta_eta_vec)
  [ksi_i_vec] -> update dpsy psy agent 4/5(ksi_i_vec)
  Constant52/1 -> update dpsy psy agent 4/1(Wij)
  [ksi_d_est_vec] -> update dpsy psy agent 4/7(ksi_d_est_vec)
  [eta_d_est_vec] -> update dpsy psy agent 4/8(eta_d_est_vec)
  psy Integrator 4/1 -> [psy_4]
  d_psy Integrator 4/1 -> [d_psy_4], psy Integrator 4/1
  [delta_ksi_vec] -> update dpsy psy agent 4/3(delta_ksi_vec)
  d_psy Integrator 5/1 -> [d_psy_5], psy Integrator 5/1
  [eta_d_est_vec] -> update dpsy psy agent 5/8(eta_d_est_vec)
  [ksi_d_est_vec] -> update dpsy psy agent 5/7(ksi_d_est_vec)
  psy Integrator 5/1 -> [psy_5]
  [delta_ksi_vec] -> update dpsy psy agent 5/3(delta_ksi_vec)
  [eta_i_vec] -> update dpsy psy agent 5/6(eta_i_vec)
  Constant54/1 -> update dpsy psy agent 5/1(Wij)
  Constant55/1 -> update dpsy psy agent 5/2(Mii)
  update dpsy psy agent 5/1(d_2_psy_5) -> d_psy Integrator 5/1
  [delta_eta_vec] -> update dpsy psy agent 5/4(delta_eta_vec)
  [ksi_i_vec] -> update dpsy psy agent 5/5(ksi_i_vec)
  [delta_ksi_vec] -> cal si agent 1/3(delta_ksi_vec)
  [ksi_d_est_vec] -> cal si agent 2/6(ksi_d_est_vec)
  [ksi_i_vec] -> cal si agent 2/5(ksi_i_vec)
  Constant56/1 -> cal si agent 2/1(Wij)
  [ksi0] -> cal si agent 2/4(ksi0)
  cal si agent 2/1(si_2) -> [si_2]
  Constant57/1 -> cal si agent 2/2(Mii)
  [delta_ksi_vec] -> cal si agent 2/3(delta_ksi_vec)
  Constant59/1 -> cal si agent 3/2(Mii)
  cal si agent 3/1(si_3) -> [si_3]
  [ksi_d_est_vec] -> cal si agent 3/6(ksi_d_est_vec)
  Constant58/1 -> cal si agent 3/1(Wij)
  [delta_ksi_vec] -> cal si agent 3/3(delta_ksi_vec)
  [ksi_i_vec] -> cal si agent 3/5(ksi_i_vec)
  [ksi0] -> cal si agent 3/4(ksi0)
  Constant60/1 -> cal si agent 4/1(Wij)
  Constant63/1 -> cal si agent 4/2(Mii)
  cal si agent 4/1(si_4) -> [si_4]
  [ksi_i_vec] -> cal si agent 4/5(ksi_i_vec)
  [ksi_d_est_vec] -> cal si agent 4/6(ksi_d_est_vec)
  [delta_ksi_vec] -> cal si agent 4/3(delta_ksi_vec)
  [ksi0] -> cal si agent 4/4(ksi0)
  [delta_ksi_vec] -> cal si agent 5/3(delta_ksi_vec)
  [ksi_d_est_vec] -> cal si agent 5/6(ksi_d_est_vec)
  [ksi0] -> cal si agent 5/4(ksi0)
  Constant65/1 -> cal si agent 5/2(Mii)
  [ksi_i_vec] -> cal si agent 5/5(ksi_i_vec)
  cal si agent 5/1(si_5) -> [si_5]
  Constant64/1 -> cal si agent 5/1(Wij)
  [delta_eta_vec] -> cal ri agent 1/3(delta_eta_vec)
  cal ri agent 2/1(ri_2) -> [ri_2]
  Constant66/1 -> cal ri agent 2/1(Wij)
  [eta_d_est_vec] -> cal ri agent 2/6(eta_d_est_vec)
  Constant67/1 -> cal ri agent 2/2(Mii)
  [eta_i_vec] -> cal ri agent 2/5(eta_i_vec)
  [eta0] -> cal ri agent 2/4(eta0)
  [delta_eta_vec] -> cal ri agent 2/3(delta_eta_vec)
  Constant68/1 -> cal ri agent 3/1(Wij)
  [delta_eta_vec] -> cal ri agent 3/3(delta_eta_vec)
  [eta_d_est_vec] -> cal ri agent 3/6(eta_d_est_vec)
  [eta_i_vec] -> cal ri agent 3/5(eta_i_vec)
  cal ri agent 3/1(ri_3) -> [ri_3]
  [eta0] -> cal ri agent 3/4(eta0)
  Constant69/1 -> cal ri agent 3/2(Mii)
  [eta_d_est_vec] -> cal ri agent 4/6(eta_d_est_vec)
  [delta_eta_vec] -> cal ri agent 4/3(delta_eta_vec)
  Constant70/1 -> cal ri agent 4/1(Wij)
  Constant71/1 -> cal ri agent 4/2(Mii)
  [eta0] -> cal ri agent 4/4(eta0)
  [eta_i_vec] -> cal ri agent 4/5(eta_i_vec)
  cal ri agent 4/1(ri_4) -> [ri_4]
  [eta_d_est_vec] -> cal ri agent 5/6(eta_d_est_vec)
  cal ri agent 5/1(ri_5) -> [ri_5]
  [eta0] -> cal ri agent 5/4(eta0)
  Constant73/1 -> cal ri agent 5/2(Mii)
  [delta_eta_vec] -> cal ri agent 5/3(delta_eta_vec)
  [eta_i_vec] -> cal ri agent 5/5(eta_i_vec)
  Constant72/1 -> cal ri agent 5/1(Wij)
  [delta_ksi_vec] -> follower tracking error agent 1/1(delta_ksi_vec)
  [delta_eta_vec] -> follower tracking error agent 1/2(delta_eta_vec)
  [delta_eta_vec] -> follower tracking error agent 2/2(delta_eta_vec)
  [delta_ksi_vec] -> follower tracking error agent 2/1(delta_ksi_vec)
  [delta_ksi_vec] -> follower tracking error agent 3/1(delta_ksi_vec)
  [delta_eta_vec] -> follower tracking error agent 3/2(delta_eta_vec)
  [delta_eta_vec] -> follower tracking error agent 4/2(delta_eta_vec)
  [delta_ksi_vec] -> follower tracking error agent 4/1(delta_ksi_vec)
  [delta_eta_vec] -> follower tracking error agent 5/2(delta_eta_vec)
  [delta_ksi_vec] -> follower tracking error agent 5/1(delta_ksi_vec)
  [delta_ksi_vec] -> To Workspace23/1
  [delta_eta_vec] -> To Workspace24/1
